simulink library "thermalCoupledCellResolution"  (R2025a)
settings: Solver=VariableStepAuto  StartTime=0.0  StopTime=10.0  RelTol=1e-3
undefined symbols (not defined in the file or in its folder): battery_builder_rtmsupport, gcbh
libraries: thermalCoupledCellResolution_lib x32
(part 2 of 3)

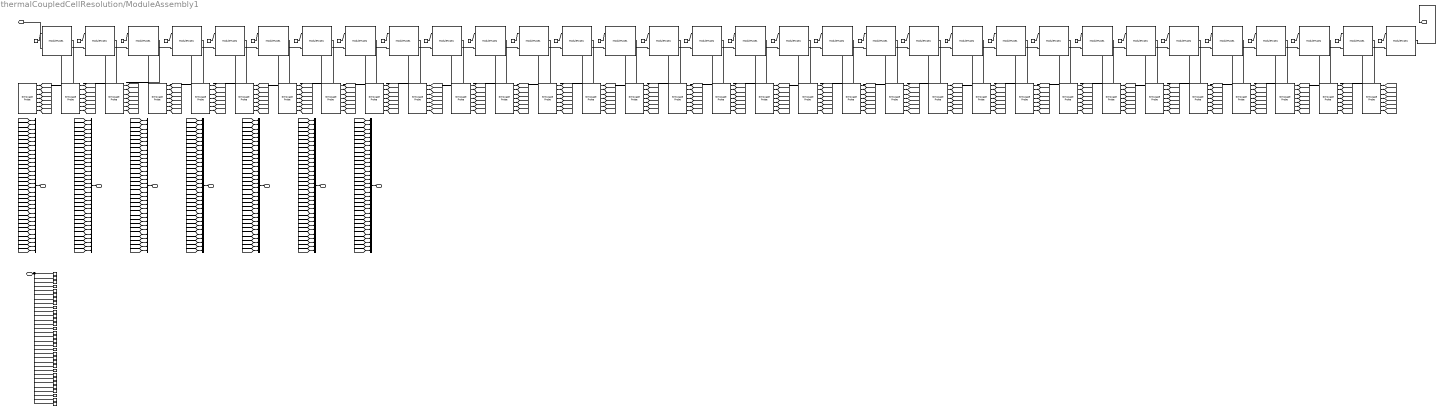
== system thermalCoupledCellResolution/ModuleAssembly1 ==
  note: Battery Modules
  note: Output Signals
  note: Thermal Boundary Conditions
  AmbH_From_1 : ConnectionLabel  Label=ambH_1
  AmbH_From_10 : ConnectionLabel  Label=ambH_10
  AmbH_From_11 : ConnectionLabel  Label=ambH_11
  AmbH_From_12 : ConnectionLabel  Label=ambH_12
  AmbH_From_13 : ConnectionLabel  Label=ambH_13
  AmbH_From_14 : ConnectionLabel  Label=ambH_14
  AmbH_From_15 : ConnectionLabel  Label=ambH_15
  AmbH_From_16 : ConnectionLabel  Label=ambH_16
  AmbH_From_17 : ConnectionLabel  Label=ambH_17
  AmbH_From_18 : ConnectionLabel  Label=ambH_18
  AmbH_From_19 : ConnectionLabel  Label=ambH_19
  AmbH_From_2 : ConnectionLabel  Label=ambH_2
  AmbH_From_20 : ConnectionLabel  Label=ambH_20
  AmbH_From_21 : ConnectionLabel  Label=ambH_21
  AmbH_From_22 : ConnectionLabel  Label=ambH_22
  AmbH_From_23 : ConnectionLabel  Label=ambH_23
  AmbH_From_24 : ConnectionLabel  Label=ambH_24
  AmbH_From_25 : ConnectionLabel  Label=ambH_25
  AmbH_From_26 : ConnectionLabel  Label=ambH_26
  AmbH_From_27 : ConnectionLabel  Label=ambH_27
  AmbH_From_28 : ConnectionLabel  Label=ambH_28
  AmbH_From_29 : ConnectionLabel  Label=ambH_29
  AmbH_From_3 : ConnectionLabel  Label=ambH_3
  AmbH_From_30 : ConnectionLabel  Label=ambH_30
  AmbH_From_31 : ConnectionLabel  Label=ambH_31
  AmbH_From_32 : ConnectionLabel  Label=ambH_32
  AmbH_From_4 : ConnectionLabel  Label=ambH_4
  AmbH_From_5 : ConnectionLabel  Label=ambH_5
  AmbH_From_6 : ConnectionLabel  Label=ambH_6
  AmbH_From_7 : ConnectionLabel  Label=ambH_7
  AmbH_From_8 : ConnectionLabel  Label=ambH_8
  AmbH_From_9 : ConnectionLabel  Label=ambH_9
  AmbH_To_1 : ConnectionLabel  Label=ambH_1
  AmbH_To_10 : ConnectionLabel  Label=ambH_10
  AmbH_To_11 : ConnectionLabel  Label=ambH_11
  AmbH_To_12 : ConnectionLabel  Label=ambH_12
  AmbH_To_13 : ConnectionLabel  Label=ambH_13
  AmbH_To_14 : ConnectionLabel  Label=ambH_14
  AmbH_To_15 : ConnectionLabel  Label=ambH_15
  AmbH_To_16 : ConnectionLabel  Label=ambH_16
  AmbH_To_17 : ConnectionLabel  Label=ambH_17
  AmbH_To_18 : ConnectionLabel  Label=ambH_18
  AmbH_To_19 : ConnectionLabel  Label=ambH_19
  AmbH_To_2 : ConnectionLabel  Label=ambH_2
  AmbH_To_20 : ConnectionLabel  Label=ambH_20
  AmbH_To_21 : ConnectionLabel  Label=ambH_21
  AmbH_To_22 : ConnectionLabel  Label=ambH_22
  AmbH_To_23 : ConnectionLabel  Label=ambH_23
  AmbH_To_24 : ConnectionLabel  Label=ambH_24
  AmbH_To_25 : ConnectionLabel  Label=ambH_25
  AmbH_To_26 : ConnectionLabel  Label=ambH_26
  AmbH_To_27 : ConnectionLabel  Label=ambH_27
  AmbH_To_28 : ConnectionLabel  Label=ambH_28
  AmbH_To_29 : ConnectionLabel  Label=ambH_29
  AmbH_To_3 : ConnectionLabel  Label=ambH_3
  AmbH_To_30 : ConnectionLabel  Label=ambH_30
  AmbH_To_31 : ConnectionLabel  Label=ambH_31
  AmbH_To_32 : ConnectionLabel  Label=ambH_32
  AmbH_To_4 : ConnectionLabel  Label=ambH_4
  AmbH_To_5 : ConnectionLabel  Label=ambH_5
  AmbH_To_6 : ConnectionLabel  Label=ambH_6
  AmbH_To_7 : ConnectionLabel  Label=ambH_7
  AmbH_To_8 : ConnectionLabel  Label=ambH_8
  AmbH_To_9 : ConnectionLabel  Label=ambH_9
  Module01 : thermalCoupledCellResolution_lib/Modules/ModuleType1  BatteryCapacityCell=Module01.BatteryCapacityCell A*hr  BatteryCapacityCellPercentDeviation=Module01.BatteryCapacityCellPercentDeviation  ExtrapolationMethodCell=simscape.enum.extrapolation.nearest  SOCBreakpointsCell=Module01.SOCBreakpointsCell  SOCBreakpointsCellPercentDeviation=Module01.SOCBreakpointsCellPercentDeviation  TemperatureBreakpointsCell=Module01.TemperatureBreakpointsCell K  TemperatureBreakpointsCellPercentDeviation=Module01.TemperatureBreakpointsCellPercentDeviation  OpenCircuitVoltageThermalCell=Module01.OpenCircuitVoltageThermalCell V  OpenCircuitVoltageThermalCellPercentDeviation=Module01.OpenCircuitVoltageThermalCellPercentDeviation  VoltageRangeCell=Module01.VoltageRangeCell V  VoltageRangeCellPercentDeviation=Module01.VoltageRangeCellPercentDeviation  ResistanceSOCBreakpointsCell=Module01.ResistanceSOCBreakpointsCell  ResistanceSOCBreakpointsCellPercentDeviation=Module01.ResistanceSOCBreakpointsCellPercentDeviation  ResistanceTemperatureBreakpointsCell=Module01.ResistanceTemperatureBreakpointsCell K  ResistanceTemperatureBreakpointsCellPercentDeviation=Module01.ResistanceTemperatureBreakpointsCellPercentDeviation  R0ThermalCell=Module01.R0ThermalCell Ohm  R0ThermalCellPercentDeviation=Module01.R0ThermalCellPercentDeviation  R1ThermalCell=Module01.R1ThermalCell Ohm  R1ThermalCellPercentDeviation=Module01.R1ThermalCellPercentDeviation  Tau1ThermalCell=Module01.Tau1ThermalCell s  Tau1ThermalCellPercentDeviation=Module01.Tau1ThermalCellPercentDeviation  BatteryThermalMassCell=Module01.BatteryThermalMassCell J/K  BatteryThermalMassCellPercentDeviation=Module01.BatteryThermalMassCellPercentDeviation  AmbientResistance=Module01.AmbientResistance K/W  P=2  S=6  socCell_specify=on  socCell_priority=High  socCell=Module01.socCell  socCell_nominal_specify=off  socCell_nominal_value=1  socCell_nominal_unit=1  batteryVoltage_specify=on  batteryVoltage_priority=None  batteryVoltage=Module01.batteryVoltage V  batteryVoltage_nominal_specify=off  batteryVoltage_nominal_value=1  batteryVoltage_nominal_unit=V  batteryCurrent_specify=on  batteryCurrent_priority=None  batteryCurrent=Module01.batteryCurrent A  batteryCurrent_nominal_specify=off  batteryCurrent_nominal_value=1  batteryCurrent_nominal_unit=A  numCycles_specify=on  numCycles_priority=High  numCycles=Module01.numCycles  numCycles_nominal_specify=off  numCycles_nominal_value=1  numCycles_nominal_unit=1  batteryTemperature_specify=on  batteryTemperature_priority=High  batteryTemperature=Module01.batteryTemperature K  batteryTemperature_nominal_specify=off  batteryTemperature_nominal_value=1  batteryTemperature_nominal_unit=K  vParallelAssembly_specify=on  vParallelAssembly_priority=None  vParallelAssembly=Module01.vParallelAssembly V  vParallelAssembly_nominal_specify=off  vParallelAssembly_nominal_value=1  vParallelAssembly_nominal_unit=V  socParallelAssembly_specify=on  socParallelAssembly_priority=None  socParallelAssembly=Module01.socParallelAssembly  socParallelAssembly_nominal_specify=off  socParallelAssembly_nominal_value=1  socParallelAssembly_nominal_unit=1
      settings: InternalSimscapePortConfiguration="{\"Bottom\":[{\"id\":\"n\",\"label\":\"-\",\"type\":\"foundation.electrical.electrical\"}],\"Left\":[{\"id\":\"AmbH\",\"label\":\"AmbH\",\"type\":\"foundation.thermal.thermal\"}],\"Right\":[],\"Top\":[{\"id\":\"p\",\"label\":\"+\",\"type\":\"foundation.electrical.electrical\"}]}"
  Module01_outputs : SimscapeProbe  BoundBlock=2  Variables="{\"batteryCurrent\":{\"Probing\":\"ON\"},\"batteryTemperature\":{\"Probing\":\"ON\"},\"batteryVoltage\":{\"Probing\":\"ON\"},\"numCycles\":{\"Probing\":\"ON\"},\"socCell\":{\"Probing\":\"ON\"},\"socParallelAssembly\":{\"Probing\":\"ON\"},\"vParallelAssembly\":{\"Probing\":\"ON\"}}"
  Module02 : thermalCoupledCellResolution_lib/Modules/ModuleType1  BatteryCapacityCell=Module02.BatteryCapacityCell A*hr  BatteryCapacityCellPercentDeviation=Module02.BatteryCapacityCellPercentDeviation  ExtrapolationMethodCell=simscape.enum.extrapolation.nearest  SOCBreakpointsCell=Module02.SOCBreakpointsCell  SOCBreakpointsCellPercentDeviation=Module02.SOCBreakpointsCellPercentDeviation  TemperatureBreakpointsCell=Module02.TemperatureBreakpointsCell K  TemperatureBreakpointsCellPercentDeviation=Module02.TemperatureBreakpointsCellPercentDeviation  OpenCircuitVoltageThermalCell=Module02.OpenCircuitVoltageThermalCell V  OpenCircuitVoltageThermalCellPercentDeviation=Module02.OpenCircuitVoltageThermalCellPercentDeviation  VoltageRangeCell=Module02.VoltageRangeCell V  VoltageRangeCellPercentDeviation=Module02.VoltageRangeCellPercentDeviation  ResistanceSOCBreakpointsCell=Module02.ResistanceSOCBreakpointsCell  ResistanceSOCBreakpointsCellPercentDeviation=Module02.ResistanceSOCBreakpointsCellPercentDeviation  ResistanceTemperatureBreakpointsCell=Module02.ResistanceTemperatureBreakpointsCell K  ResistanceTemperatureBreakpointsCellPercentDeviation=Module02.ResistanceTemperatureBreakpointsCellPercentDeviation  R0ThermalCell=Module02.R0ThermalCell Ohm  R0ThermalCellPercentDeviation=Module02.R0ThermalCellPercentDeviation  R1ThermalCell=Module02.R1ThermalCell Ohm  R1ThermalCellPercentDeviation=Module02.R1ThermalCellPercentDeviation  Tau1ThermalCell=Module02.Tau1ThermalCell s  Tau1ThermalCellPercentDeviation=Module02.Tau1ThermalCellPercentDeviation  BatteryThermalMassCell=Module02.BatteryThermalMassCell J/K  BatteryThermalMassCellPercentDeviation=Module02.BatteryThermalMassCellPercentDeviation  AmbientResistance=Module02.AmbientResistance K/W  P=2  S=6  socCell_specify=on  socCell_priority=High  socCell=Module02.socCell  socCell_nominal_specify=off  socCell_nominal_value=1  socCell_nominal_unit=1  batteryVoltage_specify=on  batteryVoltage_priority=None  batteryVoltage=Module02.batteryVoltage V  batteryVoltage_nominal_specify=off  batteryVoltage_nominal_value=1  batteryVoltage_nominal_unit=V  batteryCurrent_specify=on  batteryCurrent_priority=None  batteryCurrent=Module02.batteryCurrent A  batteryCurrent_nominal_specify=off  batteryCurrent_nominal_value=1  batteryCurrent_nominal_unit=A  numCycles_specify=on  numCycles_priority=High  numCycles=Module02.numCycles  numCycles_nominal_specify=off  numCycles_nominal_value=1  numCycles_nominal_unit=1  batteryTemperature_specify=on  batteryTemperature_priority=High  batteryTemperature=Module02.batteryTemperature K  batteryTemperature_nominal_specify=off  batteryTemperature_nominal_value=1  batteryTemperature_nominal_unit=K  vParallelAssembly_specify=on  vParallelAssembly_priority=None  vParallelAssembly=Module02.vParallelAssembly V  vParallelAssembly_nominal_specify=off  vParallelAssembly_nominal_value=1  vParallelAssembly_nominal_unit=V  socParallelAssembly_specify=on  socParallelAssembly_priority=None  socParallelAssembly=Module02.socParallelAssembly  socParallelAssembly_nominal_specify=off  socParallelAssembly_nominal_value=1  socParallelAssembly_nominal_unit=1
      settings: InternalSimscapePortConfiguration="{\"Bottom\":[{\"id\":\"n\",\"label\":\"-\",\"type\":\"foundation.electrical.electrical\"}],\"Left\":[{\"id\":\"AmbH\",\"label\":\"AmbH\",\"type\":\"foundation.thermal.thermal\"}],\"Right\":[],\"Top\":[{\"id\":\"p\",\"label\":\"+\",\"type\":\"foundation.electrical.electrical\"}]}"
  Module02_outputs : SimscapeProbe  BoundBlock=3  Variables="{\"batteryCurrent\":{\"Probing\":\"ON\"},\"batteryTemperature\":{\"Probing\":\"ON\"},\"batteryVoltage\":{\"Probing\":\"ON\"},\"numCycles\":{\"Probing\":\"ON\"},\"socCell\":{\"Probing\":\"ON\"},\"socParallelAssembly\":{\"Probing\":\"ON\"},\"vParallelAssembly\":{\"Probing\":\"ON\"}}"
  Module03 : thermalCoupledCellResolution_lib/Modules/ModuleType1  BatteryCapacityCell=Module03.BatteryCapacityCell A*hr  BatteryCapacityCellPercentDeviation=Module03.BatteryCapacityCellPercentDeviation  ExtrapolationMethodCell=simscape.enum.extrapolation.nearest  SOCBreakpointsCell=Module03.SOCBreakpointsCell  SOCBreakpointsCellPercentDeviation=Module03.SOCBreakpointsCellPercentDeviation  TemperatureBreakpointsCell=Module03.TemperatureBreakpointsCell K  TemperatureBreakpointsCellPercentDeviation=Module03.TemperatureBreakpointsCellPercentDeviation  OpenCircuitVoltageThermalCell=Module03.OpenCircuitVoltageThermalCell V  OpenCircuitVoltageThermalCellPercentDeviation=Module03.OpenCircuitVoltageThermalCellPercentDeviation  VoltageRangeCell=Module03.VoltageRangeCell V  VoltageRangeCellPercentDeviation=Module03.VoltageRangeCellPercentDeviation  ResistanceSOCBreakpointsCell=Module03.ResistanceSOCBreakpointsCell  ResistanceSOCBreakpointsCellPercentDeviation=Module03.ResistanceSOCBreakpointsCellPercentDeviation  ResistanceTemperatureBreakpointsCell=Module03.ResistanceTemperatureBreakpointsCell K  ResistanceTemperatureBreakpointsCellPercentDeviation=Module03.ResistanceTemperatureBreakpointsCellPercentDeviation  R0ThermalCell=Module03.R0ThermalCell Ohm  R0ThermalCellPercentDeviation=Module03.R0ThermalCellPercentDeviation  R1ThermalCell=Module03.R1ThermalCell Ohm  R1ThermalCellPercentDeviation=Module03.R1ThermalCellPercentDeviation  Tau1ThermalCell=Module03.Tau1ThermalCell s  Tau1ThermalCellPercentDeviation=Module03.Tau1ThermalCellPercentDeviation  BatteryThermalMassCell=Module03.BatteryThermalMassCell J/K  BatteryThermalMassCellPercentDeviation=Module03.BatteryThermalMassCellPercentDeviation  AmbientResistance=Module03.AmbientResistance K/W  P=2  S=6  socCell_specify=on  socCell_priority=High  socCell=Module03.socCell  socCell_nominal_specify=off  socCell_nominal_value=1  socCell_nominal_unit=1  batteryVoltage_specify=on  batteryVoltage_priority=None  batteryVoltage=Module03.batteryVoltage V  batteryVoltage_nominal_specify=off  batteryVoltage_nominal_value=1  batteryVoltage_nominal_unit=V  batteryCurrent_specify=on  batteryCurrent_priority=None  batteryCurrent=Module03.batteryCurrent A  batteryCurrent_nominal_specify=off  batteryCurrent_nominal_value=1  batteryCurrent_nominal_unit=A  numCycles_specify=on  numCycles_priority=High  numCycles=Module03.numCycles  numCycles_nominal_specify=off  numCycles_nominal_value=1  numCycles_nominal_unit=1  batteryTemperature_specify=on  batteryTemperature_priority=High  batteryTemperature=Module03.batteryTemperature K  batteryTemperature_nominal_specify=off  batteryTemperature_nominal_value=1  batteryTemperature_nominal_unit=K  vParallelAssembly_specify=on  vParallelAssembly_priority=None  vParallelAssembly=Module03.vParallelAssembly V  vParallelAssembly_nominal_specify=off  vParallelAssembly_nominal_value=1  vParallelAssembly_nominal_unit=V  socParallelAssembly_specify=on  socParallelAssembly_priority=None  socParallelAssembly=Module03.socParallelAssembly  socParallelAssembly_nominal_specify=off  socParallelAssembly_nominal_value=1  socParallelAssembly_nominal_unit=1
      settings: InternalSimscapePortConfiguration="{\"Bottom\":[{\"id\":\"n\",\"label\":\"-\",\"type\":\"foundation.electrical.electrical\"}],\"Left\":[{\"id\":\"AmbH\",\"label\":\"AmbH\",\"type\":\"foundation.thermal.thermal\"}],\"Right\":[],\"Top\":[{\"id\":\"p\",\"label\":\"+\",\"type\":\"foundation.electrical.electrical\"}]}"
  Module03_outputs : SimscapeProbe  BoundBlock=4  Variables="{\"batteryCurrent\":{\"Probing\":\"ON\"},\"batteryTemperature\":{\"Probing\":\"ON\"},\"batteryVoltage\":{\"Probing\":\"ON\"},\"numCycles\":{\"Probing\":\"ON\"},\"socCell\":{\"Probing\":\"ON\"},\"socParallelAssembly\":{\"Probing\":\"ON\"},\"vParallelAssembly\":{\"Probing\":\"ON\"}}"
  Module04 : thermalCoupledCellResolution_lib/Modules/ModuleType1  BatteryCapacityCell=Module04.BatteryCapacityCell A*hr  BatteryCapacityCellPercentDeviation=Module04.BatteryCapacityCellPercentDeviation  ExtrapolationMethodCell=simscape.enum.extrapolation.nearest  SOCBreakpointsCell=Module04.SOCBreakpointsCell  SOCBreakpointsCellPercentDeviation=Module04.SOCBreakpointsCellPercentDeviation  TemperatureBreakpointsCell=Module04.TemperatureBreakpointsCell K  TemperatureBreakpointsCellPercentDeviation=Module04.TemperatureBreakpointsCellPercentDeviation  OpenCircuitVoltageThermalCell=Module04.OpenCircuitVoltageThermalCell V  OpenCircuitVoltageThermalCellPercentDeviation=Module04.OpenCircuitVoltageThermalCellPercentDeviation  VoltageRangeCell=Module04.VoltageRangeCell V  VoltageRangeCellPercentDeviation=Module04.VoltageRangeCellPercentDeviation  ResistanceSOCBreakpointsCell=Module04.ResistanceSOCBreakpointsCell  ResistanceSOCBreakpointsCellPercentDeviation=Module04.ResistanceSOCBreakpointsCellPercentDeviation  ResistanceTemperatureBreakpointsCell=Module04.ResistanceTemperatureBreakpointsCell K  ResistanceTemperatureBreakpointsCellPercentDeviation=Module04.ResistanceTemperatureBreakpointsCellPercentDeviation  R0ThermalCell=Module04.R0ThermalCell Ohm  R0ThermalCellPercentDeviation=Module04.R0ThermalCellPercentDeviation  R1ThermalCell=Module04.R1ThermalCell Ohm  R1ThermalCellPercentDeviation=Module04.R1ThermalCellPercentDeviation  Tau1ThermalCell=Module04.Tau1ThermalCell s  Tau1ThermalCellPercentDeviation=Module04.Tau1ThermalCellPercentDeviation  BatteryThermalMassCell=Module04.BatteryThermalMassCell J/K  BatteryThermalMassCellPercentDeviation=Module04.BatteryThermalMassCellPercentDeviation  AmbientResistance=Module04.AmbientResistance K/W  P=2  S=6  socCell_specify=on  socCell_priority=High  socCell=Module04.socCell  socCell_nominal_specify=off  socCell_nominal_value=1  socCell_nominal_unit=1  batteryVoltage_specify=on  batteryVoltage_priority=None  batteryVoltage=Module04.batteryVoltage V  batteryVoltage_nominal_specify=off  batteryVoltage_nominal_value=1  batteryVoltage_nominal_unit=V  batteryCurrent_specify=on  batteryCurrent_priority=None  batteryCurrent=Module04.batteryCurrent A  batteryCurrent_nominal_specify=off  batteryCurrent_nominal_value=1  batteryCurrent_nominal_unit=A  numCycles_specify=on  numCycles_priority=High  numCycles=Module04.numCycles  numCycles_nominal_specify=off  numCycles_nominal_value=1  numCycles_nominal_unit=1  batteryTemperature_specify=on  batteryTemperature_priority=High  batteryTemperature=Module04.batteryTemperature K  batteryTemperature_nominal_specify=off  batteryTemperature_nominal_value=1  batteryTemperature_nominal_unit=K  vParallelAssembly_specify=on  vParallelAssembly_priority=None  vParallelAssembly=Module04.vParallelAssembly V  vParallelAssembly_nominal_specify=off  vParallelAssembly_nominal_value=1  vParallelAssembly_nominal_unit=V  socParallelAssembly_specify=on  socParallelAssembly_priority=None  socParallelAssembly=Module04.socParallelAssembly  socParallelAssembly_nominal_specify=off  socParallelAssembly_nominal_value=1  socParallelAssembly_nominal_unit=1
      settings: InternalSimscapePortConfiguration="{\"Bottom\":[{\"id\":\"n\",\"label\":\"-\",\"type\":\"foundation.electrical.electrical\"}],\"Left\":[{\"id\":\"AmbH\",\"label\":\"AmbH\",\"type\":\"foundation.thermal.thermal\"}],\"Right\":[],\"Top\":[{\"id\":\"p\",\"label\":\"+\",\"type\":\"foundation.electrical.electrical\"}]}"
  Module04_outputs : SimscapeProbe  BoundBlock=5  Variables="{\"batteryCurrent\":{\"Probing\":\"ON\"},\"batteryTemperature\":{\"Probing\":\"ON\"},\"batteryVoltage\":{\"Probing\":\"ON\"},\"numCycles\":{\"Probing\":\"ON\"},\"socCell\":{\"Probing\":\"ON\"},\"socParallelAssembly\":{\"Probing\":\"ON\"},\"vParallelAssembly\":{\"Probing\":\"ON\"}}"
  Module05 : thermalCoupledCellResolution_lib/Modules/ModuleType1  BatteryCapacityCell=Module05.BatteryCapacityCell A*hr  BatteryCapacityCellPercentDeviation=Module05.BatteryCapacityCellPercentDeviation  ExtrapolationMethodCell=simscape.enum.extrapolation.nearest  SOCBreakpointsCell=Module05.SOCBreakpointsCell  SOCBreakpointsCellPercentDeviation=Module05.SOCBreakpointsCellPercentDeviation  TemperatureBreakpointsCell=Module05.TemperatureBreakpointsCell K  TemperatureBreakpointsCellPercentDeviation=Module05.TemperatureBreakpointsCellPercentDeviation  OpenCircuitVoltageThermalCell=Module05.OpenCircuitVoltageThermalCell V  OpenCircuitVoltageThermalCellPercentDeviation=Module05.OpenCircuitVoltageThermalCellPercentDeviation  VoltageRangeCell=Module05.VoltageRangeCell V  VoltageRangeCellPercentDeviation=Module05.VoltageRangeCellPercentDeviation  ResistanceSOCBreakpointsCell=Module05.ResistanceSOCBreakpointsCell  ResistanceSOCBreakpointsCellPercentDeviation=Module05.ResistanceSOCBreakpointsCellPercentDeviation  ResistanceTemperatureBreakpointsCell=Module05.ResistanceTemperatureBreakpointsCell K  ResistanceTemperatureBreakpointsCellPercentDeviation=Module05.ResistanceTemperatureBreakpointsCellPercentDeviation  R0ThermalCell=Module05.R0ThermalCell Ohm  R0ThermalCellPercentDeviation=Module05.R0ThermalCellPercentDeviation  R1ThermalCell=Module05.R1ThermalCell Ohm  R1ThermalCellPercentDeviation=Module05.R1ThermalCellPercentDeviation  Tau1ThermalCell=Module05.Tau1ThermalCell s  Tau1ThermalCellPercentDeviation=Module05.Tau1ThermalCellPercentDeviation  BatteryThermalMassCell=Module05.BatteryThermalMassCell J/K  BatteryThermalMassCellPercentDeviation=Module05.BatteryThermalMassCellPercentDeviation  AmbientResistance=Module05.AmbientResistance K/W  P=2  S=6  socCell_specify=on  socCell_priority=High  socCell=Module05.socCell  socCell_nominal_specify=off  socCell_nominal_value=1  socCell_nominal_unit=1  batteryVoltage_specify=on  batteryVoltage_priority=None  batteryVoltage=Module05.batteryVoltage V  batteryVoltage_nominal_specify=off  batteryVoltage_nominal_value=1  batteryVoltage_nominal_unit=V  batteryCurrent_specify=on  batteryCurrent_priority=None  batteryCurrent=Module05.batteryCurrent A  batteryCurrent_nominal_specify=off  batteryCurrent_nominal_value=1  batteryCurrent_nominal_unit=A  numCycles_specify=on  numCycles_priority=High  numCycles=Module05.numCycles  numCycles_nominal_specify=off  numCycles_nominal_value=1  numCycles_nominal_unit=1  batteryTemperature_specify=on  batteryTemperature_priority=High  batteryTemperature=Module05.batteryTemperature K  batteryTemperature_nominal_specify=off  batteryTemperature_nominal_value=1  batteryTemperature_nominal_unit=K  vParallelAssembly_specify=on  vParallelAssembly_priority=None  vParallelAssembly=Module05.vParallelAssembly V  vParallelAssembly_nominal_specify=off  vParallelAssembly_nominal_value=1  vParallelAssembly_nominal_unit=V  socParallelAssembly_specify=on  socParallelAssembly_priority=None  socParallelAssembly=Module05.socParallelAssembly  socParallelAssembly_nominal_specify=off  socParallelAssembly_nominal_value=1  socParallelAssembly_nominal_unit=1
      settings: InternalSimscapePortConfiguration="{\"Bottom\":[{\"id\":\"n\",\"label\":\"-\",\"type\":\"foundation.electrical.electrical\"}],\"Left\":[{\"id\":\"AmbH\",\"label\":\"AmbH\",\"type\":\"foundation.thermal.thermal\"}],\"Right\":[],\"Top\":[{\"id\":\"p\",\"label\":\"+\",\"type\":\"foundation.electrical.electrical\"}]}"
  Module05_outputs : SimscapeProbe  BoundBlock=6  Variables="{\"batteryCurrent\":{\"Probing\":\"ON\"},\"batteryTemperature\":{\"Probing\":\"ON\"},\"batteryVoltage\":{\"Probing\":\"ON\"},\"numCycles\":{\"Probing\":\"ON\"},\"socCell\":{\"Probing\":\"ON\"},\"socParallelAssembly\":{\"Probing\":\"ON\"},\"vParallelAssembly\":{\"Probing\":\"ON\"}}"
  Module06 : thermalCoupledCellResolution_lib/Modules/ModuleType1  BatteryCapacityCell=Module06.BatteryCapacityCell A*hr  BatteryCapacityCellPercentDeviation=Module06.BatteryCapacityCellPercentDeviation  ExtrapolationMethodCell=simscape.enum.extrapolation.nearest  SOCBreakpointsCell=Module06.SOCBreakpointsCell  SOCBreakpointsCellPercentDeviation=Module06.SOCBreakpointsCellPercentDeviation  TemperatureBreakpointsCell=Module06.TemperatureBreakpointsCell K  TemperatureBreakpointsCellPercentDeviation=Module06.TemperatureBreakpointsCellPercentDeviation  OpenCircuitVoltageThermalCell=Module06.OpenCircuitVoltageThermalCell V  OpenCircuitVoltageThermalCellPercentDeviation=Module06.OpenCircuitVoltageThermalCellPercentDeviation  VoltageRangeCell=Module06.VoltageRangeCell V  VoltageRangeCellPercentDeviation=Module06.VoltageRangeCellPercentDeviation  ResistanceSOCBreakpointsCell=Module06.ResistanceSOCBreakpointsCell  ResistanceSOCBreakpointsCellPercentDeviation=Module06.ResistanceSOCBreakpointsCellPercentDeviation  ResistanceTemperatureBreakpointsCell=Module06.ResistanceTemperatureBreakpointsCell K  ResistanceTemperatureBreakpointsCellPercentDeviation=Module06.ResistanceTemperatureBreakpointsCellPercentDeviation  R0ThermalCell=Module06.R0ThermalCell Ohm  R0ThermalCellPercentDeviation=Module06.R0ThermalCellPercentDeviation  R1ThermalCell=Module06.R1ThermalCell Ohm  R1ThermalCellPercentDeviation=Module06.R1ThermalCellPercentDeviation  Tau1ThermalCell=Module06.Tau1ThermalCell s  Tau1ThermalCellPercentDeviation=Module06.Tau1ThermalCellPercentDeviation  BatteryThermalMassCell=Module06.BatteryThermalMassCell J/K  BatteryThermalMassCellPercentDeviation=Module06.BatteryThermalMassCellPercentDeviation  AmbientResistance=Module06.AmbientResistance K/W  P=2  S=6  socCell_specify=on  socCell_priority=High  socCell=Module06.socCell  socCell_nominal_specify=off  socCell_nominal_value=1  socCell_nominal_unit=1  batteryVoltage_specify=on  batteryVoltage_priority=None  batteryVoltage=Module06.batteryVoltage V  batteryVoltage_nominal_specify=off  batteryVoltage_nominal_value=1  batteryVoltage_nominal_unit=V  batteryCurrent_specify=on  batteryCurrent_priority=None  batteryCurrent=Module06.batteryCurrent A  batteryCurrent_nominal_specify=off  batteryCurrent_nominal_value=1  batteryCurrent_nominal_unit=A  numCycles_specify=on  numCycles_priority=High  numCycles=Module06.numCycles  numCycles_nominal_specify=off  numCycles_nominal_value=1  numCycles_nominal_unit=1  batteryTemperature_specify=on  batteryTemperature_priority=High  batteryTemperature=Module06.batteryTemperature K  batteryTemperature_nominal_specify=off  batteryTemperature_nominal_value=1  batteryTemperature_nominal_unit=K  vParallelAssembly_specify=on  vParallelAssembly_priority=None  vParallelAssembly=Module06.vParallelAssembly V  vParallelAssembly_nominal_specify=off  vParallelAssembly_nominal_value=1  vParallelAssembly_nominal_unit=V  socParallelAssembly_specify=on  socParallelAssembly_priority=None  socParallelAssembly=Module06.socParallelAssembly  socParallelAssembly_nominal_specify=off  socParallelAssembly_nominal_value=1  socParallelAssembly_nominal_unit=1
      settings: InternalSimscapePortConfiguration="{\"Bottom\":[{\"id\":\"n\",\"label\":\"-\",\"type\":\"foundation.electrical.electrical\"}],\"Left\":[{\"id\":\"AmbH\",\"label\":\"AmbH\",\"type\":\"foundation.thermal.thermal\"}],\"Right\":[],\"Top\":[{\"id\":\"p\",\"label\":\"+\",\"type\":\"foundation.electrical.electrical\"}]}"
  Module06_outputs : SimscapeProbe  BoundBlock=7  Variables="{\"batteryCurrent\":{\"Probing\":\"ON\"},\"batteryTemperature\":{\"Probing\":\"ON\"},\"batteryVoltage\":{\"Probing\":\"ON\"},\"numCycles\":{\"Probing\":\"ON\"},\"socCell\":{\"Probing\":\"ON\"},\"socParallelAssembly\":{\"Probing\":\"ON\"},\"vParallelAssembly\":{\"Probing\":\"ON\"}}"
  Module07 : thermalCoupledCellResolution_lib/Modules/ModuleType1  BatteryCapacityCell=Module07.BatteryCapacityCell A*hr  BatteryCapacityCellPercentDeviation=Module07.BatteryCapacityCellPercentDeviation  ExtrapolationMethodCell=simscape.enum.extrapolation.nearest  SOCBreakpointsCell=Module07.SOCBreakpointsCell  SOCBreakpointsCellPercentDeviation=Module07.SOCBreakpointsCellPercentDeviation  TemperatureBreakpointsCell=Module07.TemperatureBreakpointsCell K  TemperatureBreakpointsCellPercentDeviation=Module07.TemperatureBreakpointsCellPercentDeviation  OpenCircuitVoltageThermalCell=Module07.OpenCircuitVoltageThermalCell V  OpenCircuitVoltageThermalCellPercentDeviation=Module07.OpenCircuitVoltageThermalCellPercentDeviation  VoltageRangeCell=Module07.VoltageRangeCell V  VoltageRangeCellPercentDeviation=Module07.VoltageRangeCellPercentDeviation  ResistanceSOCBreakpointsCell=Module07.ResistanceSOCBreakpointsCell  ResistanceSOCBreakpointsCellPercentDeviation=Module07.ResistanceSOCBreakpointsCellPercentDeviation  ResistanceTemperatureBreakpointsCell=Module07.ResistanceTemperatureBreakpointsCell K  ResistanceTemperatureBreakpointsCellPercentDeviation=Module07.ResistanceTemperatureBreakpointsCellPercentDeviation  R0ThermalCell=Module07.R0ThermalCell Ohm  R0ThermalCellPercentDeviation=Module07.R0ThermalCellPercentDeviation  R1ThermalCell=Module07.R1ThermalCell Ohm  R1ThermalCellPercentDeviation=Module07.R1ThermalCellPercentDeviation  Tau1ThermalCell=Module07.Tau1ThermalCell s  Tau1ThermalCellPercentDeviation=Module07.Tau1ThermalCellPercentDeviation  BatteryThermalMassCell=Module07.BatteryThermalMassCell J/K  BatteryThermalMassCellPercentDeviation=Module07.BatteryThermalMassCellPercentDeviation  AmbientResistance=Module07.AmbientResistance K/W  P=2  S=6  socCell_specify=on  socCell_priority=High  socCell=Module07.socCell  socCell_nominal_specify=off  socCell_nominal_value=1  socCell_nominal_unit=1  batteryVoltage_specify=on  batteryVoltage_priority=None  batteryVoltage=Module07.batteryVoltage V  batteryVoltage_nominal_specify=off  batteryVoltage_nominal_value=1  batteryVoltage_nominal_unit=V  batteryCurrent_specify=on  batteryCurrent_priority=None  batteryCurrent=Module07.batteryCurrent A  batteryCurrent_nominal_specify=off  batteryCurrent_nominal_value=1  batteryCurrent_nominal_unit=A  numCycles_specify=on  numCycles_priority=High  numCycles=Module07.numCycles  numCycles_nominal_specify=off  numCycles_nominal_value=1  numCycles_nominal_unit=1  batteryTemperature_specify=on  batteryTemperature_priority=High  batteryTemperature=Module07.batteryTemperature K  batteryTemperature_nominal_specify=off  batteryTemperature_nominal_value=1  batteryTemperature_nominal_unit=K  vParallelAssembly_specify=on  vParallelAssembly_priority=None  vParallelAssembly=Module07.vParallelAssembly V  vParallelAssembly_nominal_specify=off  vParallelAssembly_nominal_value=1  vParallelAssembly_nominal_unit=V  socParallelAssembly_specify=on  socParallelAssembly_priority=None  socParallelAssembly=Module07.socParallelAssembly  socParallelAssembly_nominal_specify=off  socParallelAssembly_nominal_value=1  socParallelAssembly_nominal_unit=1
      settings: InternalSimscapePortConfiguration="{\"Bottom\":[{\"id\":\"n\",\"label\":\"-\",\"type\":\"foundation.electrical.electrical\"}],\"Left\":[{\"id\":\"AmbH\",\"label\":\"AmbH\",\"type\":\"foundation.thermal.thermal\"}],\"Right\":[],\"Top\":[{\"id\":\"p\",\"label\":\"+\",\"type\":\"foundation.electrical.electrical\"}]}"
  Module07_outputs : SimscapeProbe  BoundBlock=8  Variables="{\"batteryCurrent\":{\"Probing\":\"ON\"},\"batteryTemperature\":{\"Probing\":\"ON\"},\"batteryVoltage\":{\"Probing\":\"ON\"},\"numCycles\":{\"Probing\":\"ON\"},\"socCell\":{\"Probing\":\"ON\"},\"socParallelAssembly\":{\"Probing\":\"ON\"},\"vParallelAssembly\":{\"Probing\":\"ON\"}}"
  Module08 : thermalCoupledCellResolution_lib/Modules/ModuleType1  BatteryCapacityCell=Module08.BatteryCapacityCell A*hr  BatteryCapacityCellPercentDeviation=Module08.BatteryCapacityCellPercentDeviation  ExtrapolationMethodCell=simscape.enum.extrapolation.nearest  SOCBreakpointsCell=Module08.SOCBreakpointsCell  SOCBreakpointsCellPercentDeviation=Module08.SOCBreakpointsCellPercentDeviation  TemperatureBreakpointsCell=Module08.TemperatureBreakpointsCell K  TemperatureBreakpointsCellPercentDeviation=Module08.TemperatureBreakpointsCellPercentDeviation  OpenCircuitVoltageThermalCell=Module08.OpenCircuitVoltageThermalCell V  OpenCircuitVoltageThermalCellPercentDeviation=Module08.OpenCircuitVoltageThermalCellPercentDeviation  VoltageRangeCell=Module08.VoltageRangeCell V  VoltageRangeCellPercentDeviation=Module08.VoltageRangeCellPercentDeviation  ResistanceSOCBreakpointsCell=Module08.ResistanceSOCBreakpointsCell  ResistanceSOCBreakpointsCellPercentDeviation=Module08.ResistanceSOCBreakpointsCellPercentDeviation  ResistanceTemperatureBreakpointsCell=Module08.ResistanceTemperatureBreakpointsCell K  ResistanceTemperatureBreakpointsCellPercentDeviation=Module08.ResistanceTemperatureBreakpointsCellPercentDeviation  R0ThermalCell=Module08.R0ThermalCell Ohm  R0ThermalCellPercentDeviation=Module08.R0ThermalCellPercentDeviation  R1ThermalCell=Module08.R1ThermalCell Ohm  R1ThermalCellPercentDeviation=Module08.R1ThermalCellPercentDeviation  Tau1ThermalCell=Module08.Tau1ThermalCell s  Tau1ThermalCellPercentDeviation=Module08.Tau1ThermalCellPercentDeviation  BatteryThermalMassCell=Module08.BatteryThermalMassCell J/K  BatteryThermalMassCellPercentDeviation=Module08.BatteryThermalMassCellPercentDeviation  AmbientResistance=Module08.AmbientResistance K/W  P=2  S=6  socCell_specify=on  socCell_priority=High  socCell=Module08.socCell  socCell_nominal_specify=off  socCell_nominal_value=1  socCell_nominal_unit=1  batteryVoltage_specify=on  batteryVoltage_priority=None  batteryVoltage=Module08.batteryVoltage V  batteryVoltage_nominal_specify=off  batteryVoltage_nominal_value=1  batteryVoltage_nominal_unit=V  batteryCurrent_specify=on  batteryCurrent_priority=None  batteryCurrent=Module08.batteryCurrent A  batteryCurrent_nominal_specify=off  batteryCurrent_nominal_value=1  batteryCurrent_nominal_unit=A  numCycles_specify=on  numCycles_priority=High  numCycles=Module08.numCycles  numCycles_nominal_specify=off  numCycles_nominal_value=1  numCycles_nominal_unit=1  batteryTemperature_specify=on  batteryTemperature_priority=High  batteryTemperature=Module08.batteryTemperature K  batteryTemperature_nominal_specify=off  batteryTemperature_nominal_value=1  batteryTemperature_nominal_unit=K  vParallelAssembly_specify=on  vParallelAssembly_priority=None  vParallelAssembly=Module08.vParallelAssembly V  vParallelAssembly_nominal_specify=off  vParallelAssembly_nominal_value=1  vParallelAssembly_nominal_unit=V  socParallelAssembly_specify=on  socParallelAssembly_priority=None  socParallelAssembly=Module08.socParallelAssembly  socParallelAssembly_nominal_specify=off  socParallelAssembly_nominal_value=1  socParallelAssembly_nominal_unit=1
      settings: InternalSimscapePortConfiguration="{\"Bottom\":[{\"id\":\"n\",\"label\":\"-\",\"type\":\"foundation.electrical.electrical\"}],\"Left\":[{\"id\":\"AmbH\",\"label\":\"AmbH\",\"type\":\"foundation.thermal.thermal\"}],\"Right\":[],\"Top\":[{\"id\":\"p\",\"label\":\"+\",\"type\":\"foundation.electrical.electrical\"}]}"
  Module08_outputs : SimscapeProbe  BoundBlock=9  Variables="{\"batteryCurrent\":{\"Probing\":\"ON\"},\"batteryTemperature\":{\"Probing\":\"ON\"},\"batteryVoltage\":{\"Probing\":\"ON\"},\"numCycles\":{\"Probing\":\"ON\"},\"socCell\":{\"Probing\":\"ON\"},\"socParallelAssembly\":{\"Probing\":\"ON\"},\"vParallelAssembly\":{\"Probing\":\"ON\"}}"
  Module09 : thermalCoupledCellResolution_lib/Modules/ModuleType1  BatteryCapacityCell=Module09.BatteryCapacityCell A*hr  BatteryCapacityCellPercentDeviation=Module09.BatteryCapacityCellPercentDeviation  ExtrapolationMethodCell=simscape.enum.extrapolation.nearest  SOCBreakpointsCell=Module09.SOCBreakpointsCell  SOCBreakpointsCellPercentDeviation=Module09.SOCBreakpointsCellPercentDeviation  TemperatureBreakpointsCell=Module09.TemperatureBreakpointsCell K  TemperatureBreakpointsCellPercentDeviation=Module09.TemperatureBreakpointsCellPercentDeviation  OpenCircuitVoltageThermalCell=Module09.OpenCircuitVoltageThermalCell V  OpenCircuitVoltageThermalCellPercentDeviation=Module09.OpenCircuitVoltageThermalCellPercentDeviation  VoltageRangeCell=Module09.VoltageRangeCell V  VoltageRangeCellPercentDeviation=Module09.VoltageRangeCellPercentDeviation  ResistanceSOCBreakpointsCell=Module09.ResistanceSOCBreakpointsCell  ResistanceSOCBreakpointsCellPercentDeviation=Module09.ResistanceSOCBreakpointsCellPercentDeviation  ResistanceTemperatureBreakpointsCell=Module09.ResistanceTemperatureBreakpointsCell K  ResistanceTemperatureBreakpointsCellPercentDeviation=Module09.ResistanceTemperatureBreakpointsCellPercentDeviation  R0ThermalCell=Module09.R0ThermalCell Ohm  R0ThermalCellPercentDeviation=Module09.R0ThermalCellPercentDeviation  R1ThermalCell=Module09.R1ThermalCell Ohm  R1ThermalCellPercentDeviation=Module09.R1ThermalCellPercentDeviation  Tau1ThermalCell=Module09.Tau1ThermalCell s  Tau1ThermalCellPercentDeviation=Module09.Tau1ThermalCellPercentDeviation  BatteryThermalMassCell=Module09.BatteryThermalMassCell J/K  BatteryThermalMassCellPercentDeviation=Module09.BatteryThermalMassCellPercentDeviation  AmbientResistance=Module09.AmbientResistance K/W  P=2  S=6  socCell_specify=on  socCell_priority=High  socCell=Module09.socCell  socCell_nominal_specify=off  socCell_nominal_value=1  socCell_nominal_unit=1  batteryVoltage_specify=on  batteryVoltage_priority=None  batteryVoltage=Module09.batteryVoltage V  batteryVoltage_nominal_specify=off  batteryVoltage_nominal_value=1  batteryVoltage_nominal_unit=V  batteryCurrent_specify=on  batteryCurrent_priority=None  batteryCurrent=Module09.batteryCurrent A  batteryCurrent_nominal_specify=off  batteryCurrent_nominal_value=1  batteryCurrent_nominal_unit=A  numCycles_specify=on  numCycles_priority=High  numCycles=Module09.numCycles  numCycles_nominal_specify=off  numCycles_nominal_value=1  numCycles_nominal_unit=1  batteryTemperature_specify=on  batteryTemperature_priority=High  batteryTemperature=Module09.batteryTemperature K  batteryTemperature_nominal_specify=off  batteryTemperature_nominal_value=1  batteryTemperature_nominal_unit=K  vParallelAssembly_specify=on  vParallelAssembly_priority=None  vParallelAssembly=Module09.vParallelAssembly V  vParallelAssembly_nominal_specify=off  vParallelAssembly_nominal_value=1  vParallelAssembly_nominal_unit=V  socParallelAssembly_specify=on  socParallelAssembly_priority=None  socParallelAssembly=Module09.socParallelAssembly  socParallelAssembly_nominal_specify=off  socParallelAssembly_nominal_value=1  socParallelAssembly_nominal_unit=1
      settings: InternalSimscapePortConfiguration="{\"Bottom\":[{\"id\":\"n\",\"label\":\"-\",\"type\":\"foundation.electrical.electrical\"}],\"Left\":[{\"id\":\"AmbH\",\"label\":\"AmbH\",\"type\":\"foundation.thermal.thermal\"}],\"Right\":[],\"Top\":[{\"id\":\"p\",\"label\":\"+\",\"type\":\"foundation.electrical.electrical\"}]}"
  Module09_outputs : SimscapeProbe  BoundBlock=10  Variables="{\"batteryCurrent\":{\"Probing\":\"ON\"},\"batteryTemperature\":{\"Probing\":\"ON\"},\"batteryVoltage\":{\"Probing\":\"ON\"},\"numCycles\":{\"Probing\":\"ON\"},\"socCell\":{\"Probing\":\"ON\"},\"socParallelAssembly\":{\"Probing\":\"ON\"},\"vParallelAssembly\":{\"Probing\":\"ON\"}}"
  Module10 : thermalCoupledCellResolution_lib/Modules/ModuleType1  BatteryCapacityCell=Module10.BatteryCapacityCell A*hr  BatteryCapacityCellPercentDeviation=Module10.BatteryCapacityCellPercentDeviation  ExtrapolationMethodCell=simscape.enum.extrapolation.nearest  SOCBreakpointsCell=Module10.SOCBreakpointsCell  SOCBreakpointsCellPercentDeviation=Module10.SOCBreakpointsCellPercentDeviation  TemperatureBreakpointsCell=Module10.TemperatureBreakpointsCell K  TemperatureBreakpointsCellPercentDeviation=Module10.TemperatureBreakpointsCellPercentDeviation  OpenCircuitVoltageThermalCell=Module10.OpenCircuitVoltageThermalCell V  OpenCircuitVoltageThermalCellPercentDeviation=Module10.OpenCircuitVoltageThermalCellPercentDeviation  VoltageRangeCell=Module10.VoltageRangeCell V  VoltageRangeCellPercentDeviation=Module10.VoltageRangeCellPercentDeviation  ResistanceSOCBreakpointsCell=Module10.ResistanceSOCBreakpointsCell  ResistanceSOCBreakpointsCellPercentDeviation=Module10.ResistanceSOCBreakpointsCellPercentDeviation  ResistanceTemperatureBreakpointsCell=Module10.ResistanceTemperatureBreakpointsCell K  ResistanceTemperatureBreakpointsCellPercentDeviation=Module10.ResistanceTemperatureBreakpointsCellPercentDeviation  R0ThermalCell=Module10.R0ThermalCell Ohm  R0ThermalCellPercentDeviation=Module10.R0ThermalCellPercentDeviation  R1ThermalCell=Module10.R1ThermalCell Ohm  R1ThermalCellPercentDeviation=Module10.R1ThermalCellPercentDeviation  Tau1ThermalCell=Module10.Tau1ThermalCell s  Tau1ThermalCellPercentDeviation=Module10.Tau1ThermalCellPercentDeviation  BatteryThermalMassCell=Module10.BatteryThermalMassCell J/K  BatteryThermalMassCellPercentDeviation=Module10.BatteryThermalMassCellPercentDeviation  AmbientResistance=Module10.AmbientResistance K/W  P=2  S=6  socCell_specify=on  socCell_priority=High  socCell=Module10.socCell  socCell_nominal_specify=off  socCell_nominal_value=1  socCell_nominal_unit=1  batteryVoltage_specify=on  batteryVoltage_priority=None  batteryVoltage=Module10.batteryVoltage V  batteryVoltage_nominal_specify=off  batteryVoltage_nominal_value=1  batteryVoltage_nominal_unit=V  batteryCurrent_specify=on  batteryCurrent_priority=None  batteryCurrent=Module10.batteryCurrent A  batteryCurrent_nominal_specify=off  batteryCurrent_nominal_value=1  batteryCurrent_nominal_unit=A  numCycles_specify=on  numCycles_priority=High  numCycles=Module10.numCycles  numCycles_nominal_specify=off  numCycles_nominal_value=1  numCycles_nominal_unit=1  batteryTemperature_specify=on  batteryTemperature_priority=High  batteryTemperature=Module10.batteryTemperature K  batteryTemperature_nominal_specify=off  batteryTemperature_nominal_value=1  batteryTemperature_nominal_unit=K  vParallelAssembly_specify=on  vParallelAssembly_priority=None  vParallelAssembly=Module10.vParallelAssembly V  vParallelAssembly_nominal_specify=off  vParallelAssembly_nominal_value=1  vParallelAssembly_nominal_unit=V  socParallelAssembly_specify=on  socParallelAssembly_priority=None  socParallelAssembly=Module10.socParallelAssembly  socParallelAssembly_nominal_specify=off  socParallelAssembly_nominal_value=1  socParallelAssembly_nominal_unit=1
      settings: InternalSimscapePortConfiguration="{\"Bottom\":[{\"id\":\"n\",\"label\":\"-\",\"type\":\"foundation.electrical.electrical\"}],\"Left\":[{\"id\":\"AmbH\",\"label\":\"AmbH\",\"type\":\"foundation.thermal.thermal\"}],\"Right\":[],\"Top\":[{\"id\":\"p\",\"label\":\"+\",\"type\":\"foundation.electrical.electrical\"}]}"
  Module10_outputs : SimscapeProbe  BoundBlock=11  Variables="{\"batteryCurrent\":{\"Probing\":\"ON\"},\"batteryTemperature\":{\"Probing\":\"ON\"},\"batteryVoltage\":{\"Probing\":\"ON\"},\"numCycles\":{\"Probing\":\"ON\"},\"socCell\":{\"Probing\":\"ON\"},\"socParallelAssembly\":{\"Probing\":\"ON\"},\"vParallelAssembly\":{\"Probing\":\"ON\"}}"
  Module11 : thermalCoupledCellResolution_lib/Modules/ModuleType1  BatteryCapacityCell=Module11.BatteryCapacityCell A*hr  BatteryCapacityCellPercentDeviation=Module11.BatteryCapacityCellPercentDeviation  ExtrapolationMethodCell=simscape.enum.extrapolation.nearest  SOCBreakpointsCell=Module11.SOCBreakpointsCell  SOCBreakpointsCellPercentDeviation=Module11.SOCBreakpointsCellPercentDeviation  TemperatureBreakpointsCell=Module11.TemperatureBreakpointsCell K  TemperatureBreakpointsCellPercentDeviation=Module11.TemperatureBreakpointsCellPercentDeviation  OpenCircuitVoltageThermalCell=Module11.OpenCircuitVoltageThermalCell V  OpenCircuitVoltageThermalCellPercentDeviation=Module11.OpenCircuitVoltageThermalCellPercentDeviation  VoltageRangeCell=Module11.VoltageRangeCell V  VoltageRangeCellPercentDeviation=Module11.VoltageRangeCellPercentDeviation  ResistanceSOCBreakpointsCell=Module11.ResistanceSOCBreakpointsCell  ResistanceSOCBreakpointsCellPercentDeviation=Module11.ResistanceSOCBreakpointsCellPercentDeviation  ResistanceTemperatureBreakpointsCell=Module11.ResistanceTemperatureBreakpointsCell K  ResistanceTemperatureBreakpointsCellPercentDeviation=Module11.ResistanceTemperatureBreakpointsCellPercentDeviation  R0ThermalCell=Module11.R0ThermalCell Ohm  R0ThermalCellPercentDeviation=Module11.R0ThermalCellPercentDeviation  R1ThermalCell=Module11.R1ThermalCell Ohm  R1ThermalCellPercentDeviation=Module11.R1ThermalCellPercentDeviation  Tau1ThermalCell=Module11.Tau1ThermalCell s  Tau1ThermalCellPercentDeviation=Module11.Tau1ThermalCellPercentDeviation  BatteryThermalMassCell=Module11.BatteryThermalMassCell J/K  BatteryThermalMassCellPercentDeviation=Module11.BatteryThermalMassCellPercentDeviation  AmbientResistance=Module11.AmbientResistance K/W  P=2  S=6  socCell_specify=on  socCell_priority=High  socCell=Module11.socCell  socCell_nominal_specify=off  socCell_nominal_value=1  socCell_nominal_unit=1  batteryVoltage_specify=on  batteryVoltage_priority=None  batteryVoltage=Module11.batteryVoltage V  batteryVoltage_nominal_specify=off  batteryVoltage_nominal_value=1  batteryVoltage_nominal_unit=V  batteryCurrent_specify=on  batteryCurrent_priority=None  batteryCurrent=Module11.batteryCurrent A  batteryCurrent_nominal_specify=off  batteryCurrent_nominal_value=1  batteryCurrent_nominal_unit=A  numCycles_specify=on  numCycles_priority=High  numCycles=Module11.numCycles  numCycles_nominal_specify=off  numCycles_nominal_value=1  numCycles_nominal_unit=1  batteryTemperature_specify=on  batteryTemperature_priority=High  batteryTemperature=Module11.batteryTemperature K  batteryTemperature_nominal_specify=off  batteryTemperature_nominal_value=1  batteryTemperature_nominal_unit=K  vParallelAssembly_specify=on  vParallelAssembly_priority=None  vParallelAssembly=Module11.vParallelAssembly V  vParallelAssembly_nominal_specify=off  vParallelAssembly_nominal_value=1  vParallelAssembly_nominal_unit=V  socParallelAssembly_specify=on  socParallelAssembly_priority=None  socParallelAssembly=Module11.socParallelAssembly  socParallelAssembly_nominal_specify=off  socParallelAssembly_nominal_value=1  socParallelAssembly_nominal_unit=1
      settings: InternalSimscapePortConfiguration="{\"Bottom\":[{\"id\":\"n\",\"label\":\"-\",\"type\":\"foundation.electrical.electrical\"}],\"Left\":[{\"id\":\"AmbH\",\"label\":\"AmbH\",\"type\":\"foundation.thermal.thermal\"}],\"Right\":[],\"Top\":[{\"id\":\"p\",\"label\":\"+\",\"type\":\"foundation.electrical.electrical\"}]}"
  Module11_outputs : SimscapeProbe  BoundBlock=12  Variables="{\"batteryCurrent\":{\"Probing\":\"ON\"},\"batteryTemperature\":{\"Probing\":\"ON\"},\"batteryVoltage\":{\"Probing\":\"ON\"},\"numCycles\":{\"Probing\":\"ON\"},\"socCell\":{\"Probing\":\"ON\"},\"socParallelAssembly\":{\"Probing\":\"ON\"},\"vParallelAssembly\":{\"Probing\":\"ON\"}}"
  Module12 : thermalCoupledCellResolution_lib/Modules/ModuleType1  BatteryCapacityCell=Module12.BatteryCapacityCell A*hr  BatteryCapacityCellPercentDeviation=Module12.BatteryCapacityCellPercentDeviation  ExtrapolationMethodCell=simscape.enum.extrapolation.nearest  SOCBreakpointsCell=Module12.SOCBreakpointsCell  SOCBreakpointsCellPercentDeviation=Module12.SOCBreakpointsCellPercentDeviation  TemperatureBreakpointsCell=Module12.TemperatureBreakpointsCell K  TemperatureBreakpointsCellPercentDeviation=Module12.TemperatureBreakpointsCellPercentDeviation  OpenCircuitVoltageThermalCell=Module12.OpenCircuitVoltageThermalCell V  OpenCircuitVoltageThermalCellPercentDeviation=Module12.OpenCircuitVoltageThermalCellPercentDeviation  VoltageRangeCell=Module12.VoltageRangeCell V  VoltageRangeCellPercentDeviation=Module12.VoltageRangeCellPercentDeviation  ResistanceSOCBreakpointsCell=Module12.ResistanceSOCBreakpointsCell  ResistanceSOCBreakpointsCellPercentDeviation=Module12.ResistanceSOCBreakpointsCellPercentDeviation  ResistanceTemperatureBreakpointsCell=Module12.ResistanceTemperatureBreakpointsCell K  ResistanceTemperatureBreakpointsCellPercentDeviation=Module12.ResistanceTemperatureBreakpointsCellPercentDeviation  R0ThermalCell=Module12.R0ThermalCell Ohm  R0ThermalCellPercentDeviation=Module12.R0ThermalCellPercentDeviation  R1ThermalCell=Module12.R1ThermalCell Ohm  R1ThermalCellPercentDeviation=Module12.R1ThermalCellPercentDeviation  Tau1ThermalCell=Module12.Tau1ThermalCell s  Tau1ThermalCellPercentDeviation=Module12.Tau1ThermalCellPercentDeviation  BatteryThermalMassCell=Module12.BatteryThermalMassCell J/K  BatteryThermalMassCellPercentDeviation=Module12.BatteryThermalMassCellPercentDeviation  AmbientResistance=Module12.AmbientResistance K/W  P=2  S=6  socCell_specify=on  socCell_priority=High  socCell=Module12.socCell  socCell_nominal_specify=off  socCell_nominal_value=1  socCell_nominal_unit=1  batteryVoltage_specify=on  batteryVoltage_priority=None  batteryVoltage=Module12.batteryVoltage V  batteryVoltage_nominal_specify=off  batteryVoltage_nominal_value=1  batteryVoltage_nominal_unit=V  batteryCurrent_specify=on  batteryCurrent_priority=None  batteryCurrent=Module12.batteryCurrent A  batteryCurrent_nominal_specify=off  batteryCurrent_nominal_value=1  batteryCurrent_nominal_unit=A  numCycles_specify=on  numCycles_priority=High  numCycles=Module12.numCycles  numCycles_nominal_specify=off  numCycles_nominal_value=1  numCycles_nominal_unit=1  batteryTemperature_specify=on  batteryTemperature_priority=High  batteryTemperature=Module12.batteryTemperature K  batteryTemperature_nominal_specify=off  batteryTemperature_nominal_value=1  batteryTemperature_nominal_unit=K  vParallelAssembly_specify=on  vParallelAssembly_priority=None  vParallelAssembly=Module12.vParallelAssembly V  vParallelAssembly_nominal_specify=off  vParallelAssembly_nominal_value=1  vParallelAssembly_nominal_unit=V  socParallelAssembly_specify=on  socParallelAssembly_priority=None  socParallelAssembly=Module12.socParallelAssembly  socParallelAssembly_nominal_specify=off  socParallelAssembly_nominal_value=1  socParallelAssembly_nominal_unit=1
      settings: InternalSimscapePortConfiguration="{\"Bottom\":[{\"id\":\"n\",\"label\":\"-\",\"type\":\"foundation.electrical.electrical\"}],\"Left\":[{\"id\":\"AmbH\",\"label\":\"AmbH\",\"type\":\"foundation.thermal.thermal\"}],\"Right\":[],\"Top\":[{\"id\":\"p\",\"label\":\"+\",\"type\":\"foundation.electrical.electrical\"}]}"
  Module12_outputs : SimscapeProbe  BoundBlock=13  Variables="{\"batteryCurrent\":{\"Probing\":\"ON\"},\"batteryTemperature\":{\"Probing\":\"ON\"},\"batteryVoltage\":{\"Probing\":\"ON\"},\"numCycles\":{\"Probing\":\"ON\"},\"socCell\":{\"Probing\":\"ON\"},\"socParallelAssembly\":{\"Probing\":\"ON\"},\"vParallelAssembly\":{\"Probing\":\"ON\"}}"
  Module13 : thermalCoupledCellResolution_lib/Modules/ModuleType1  BatteryCapacityCell=Module13.BatteryCapacityCell A*hr  BatteryCapacityCellPercentDeviation=Module13.BatteryCapacityCellPercentDeviation  ExtrapolationMethodCell=simscape.enum.extrapolation.nearest  SOCBreakpointsCell=Module13.SOCBreakpointsCell  SOCBreakpointsCellPercentDeviation=Module13.SOCBreakpointsCellPercentDeviation  TemperatureBreakpointsCell=Module13.TemperatureBreakpointsCell K  TemperatureBreakpointsCellPercentDeviation=Module13.TemperatureBreakpointsCellPercentDeviation  OpenCircuitVoltageThermalCell=Module13.OpenCircuitVoltageThermalCell V  OpenCircuitVoltageThermalCellPercentDeviation=Module13.OpenCircuitVoltageThermalCellPercentDeviation  VoltageRangeCell=Module13.VoltageRangeCell V  VoltageRangeCellPercentDeviation=Module13.VoltageRangeCellPercentDeviation  ResistanceSOCBreakpointsCell=Module13.ResistanceSOCBreakpointsCell  ResistanceSOCBreakpointsCellPercentDeviation=Module13.ResistanceSOCBreakpointsCellPercentDeviation  ResistanceTemperatureBreakpointsCell=Module13.ResistanceTemperatureBreakpointsCell K  ResistanceTemperatureBreakpointsCellPercentDeviation=Module13.ResistanceTemperatureBreakpointsCellPercentDeviation  R0ThermalCell=Module13.R0ThermalCell Ohm  R0ThermalCellPercentDeviation=Module13.R0ThermalCellPercentDeviation  R1ThermalCell=Module13.R1ThermalCell Ohm  R1ThermalCellPercentDeviation=Module13.R1ThermalCellPercentDeviation  Tau1ThermalCell=Module13.Tau1ThermalCell s  Tau1ThermalCellPercentDeviation=Module13.Tau1ThermalCellPercentDeviation  BatteryThermalMassCell=Module13.BatteryThermalMassCell J/K  BatteryThermalMassCellPercentDeviation=Module13.BatteryThermalMassCellPercentDeviation  AmbientResistance=Module13.AmbientResistance K/W  P=2  S=6  socCell_specify=on  socCell_priority=High  socCell=Module13.socCell  socCell_nominal_specify=off  socCell_nominal_value=1  socCell_nominal_unit=1  batteryVoltage_specify=on  batteryVoltage_priority=None  batteryVoltage=Module13.batteryVoltage V  batteryVoltage_nominal_specify=off  batteryVoltage_nominal_value=1  batteryVoltage_nominal_unit=V  batteryCurrent_specify=on  batteryCurrent_priority=None  batteryCurrent=Module13.batteryCurrent A  batteryCurrent_nominal_specify=off  batteryCurrent_nominal_value=1  batteryCurrent_nominal_unit=A  numCycles_specify=on  numCycles_priority=High  numCycles=Module13.numCycles  numCycles_nominal_specify=off  numCycles_nominal_value=1  numCycles_nominal_unit=1  batteryTemperature_specify=on  batteryTemperature_priority=High  batteryTemperature=Module13.batteryTemperature K  batteryTemperature_nominal_specify=off  batteryTemperature_nominal_value=1  batteryTemperature_nominal_unit=K  vParallelAssembly_specify=on  vParallelAssembly_priority=None  vParallelAssembly=Module13.vParallelAssembly V  vParallelAssembly_nominal_specify=off  vParallelAssembly_nominal_value=1  vParallelAssembly_nominal_unit=V  socParallelAssembly_specify=on  socParallelAssembly_priority=None  socParallelAssembly=Module13.socParallelAssembly  socParallelAssembly_nominal_specify=off  socParallelAssembly_nominal_value=1  socParallelAssembly_nominal_unit=1
      settings: InternalSimscapePortConfiguration="{\"Bottom\":[{\"id\":\"n\",\"label\":\"-\",\"type\":\"foundation.electrical.electrical\"}],\"Left\":[{\"id\":\"AmbH\",\"label\":\"AmbH\",\"type\":\"foundation.thermal.thermal\"}],\"Right\":[],\"Top\":[{\"id\":\"p\",\"label\":\"+\",\"type\":\"foundation.electrical.electrical\"}]}"
  Module13_outputs : SimscapeProbe  BoundBlock=14  Variables="{\"batteryCurrent\":{\"Probing\":\"ON\"},\"batteryTemperature\":{\"Probing\":\"ON\"},\"batteryVoltage\":{\"Probing\":\"ON\"},\"numCycles\":{\"Probing\":\"ON\"},\"socCell\":{\"Probing\":\"ON\"},\"socParallelAssembly\":{\"Probing\":\"ON\"},\"vParallelAssembly\":{\"Probing\":\"ON\"}}"
  Module14 : thermalCoupledCellResolution_lib/Modules/ModuleType1  BatteryCapacityCell=Module14.BatteryCapacityCell A*hr  BatteryCapacityCellPercentDeviation=Module14.BatteryCapacityCellPercentDeviation  ExtrapolationMethodCell=simscape.enum.extrapolation.nearest  SOCBreakpointsCell=Module14.SOCBreakpointsCell  SOCBreakpointsCellPercentDeviation=Module14.SOCBreakpointsCellPercentDeviation  TemperatureBreakpointsCell=Module14.TemperatureBreakpointsCell K  TemperatureBreakpointsCellPercentDeviation=Module14.TemperatureBreakpointsCellPercentDeviation  OpenCircuitVoltageThermalCell=Module14.OpenCircuitVoltageThermalCell V  OpenCircuitVoltageThermalCellPercentDeviation=Module14.OpenCircuitVoltageThermalCellPercentDeviation  VoltageRangeCell=Module14.VoltageRangeCell V  VoltageRangeCellPercentDeviation=Module14.VoltageRangeCellPercentDeviation  ResistanceSOCBreakpointsCell=Module14.ResistanceSOCBreakpointsCell  ResistanceSOCBreakpointsCellPercentDeviation=Module14.ResistanceSOCBreakpointsCellPercentDeviation  ResistanceTemperatureBreakpointsCell=Module14.ResistanceTemperatureBreakpointsCell K  ResistanceTemperatureBreakpointsCellPercentDeviation=Module14.ResistanceTemperatureBreakpointsCellPercentDeviation  R0ThermalCell=Module14.R0ThermalCell Ohm  R0ThermalCellPercentDeviation=Module14.R0ThermalCellPercentDeviation  R1ThermalCell=Module14.R1ThermalCell Ohm  R1ThermalCellPercentDeviation=Module14.R1ThermalCellPercentDeviation  Tau1ThermalCell=Module14.Tau1ThermalCell s  Tau1ThermalCellPercentDeviation=Module14.Tau1ThermalCellPercentDeviation  BatteryThermalMassCell=Module14.BatteryThermalMassCell J/K  BatteryThermalMassCellPercentDeviation=Module14.BatteryThermalMassCellPercentDeviation  AmbientResistance=Module14.AmbientResistance K/W  P=2  S=6  socCell_specify=on  socCell_priority=High  socCell=Module14.socCell  socCell_nominal_specify=off  socCell_nominal_value=1  socCell_nominal_unit=1  batteryVoltage_specify=on  batteryVoltage_priority=None  batteryVoltage=Module14.batteryVoltage V  batteryVoltage_nominal_specify=off  batteryVoltage_nominal_value=1  batteryVoltage_nominal_unit=V  batteryCurrent_specify=on  batteryCurrent_priority=None  batteryCurrent=Module14.batteryCurrent A  batteryCurrent_nominal_specify=off  batteryCurrent_nominal_value=1  batteryCurrent_nominal_unit=A  numCycles_specify=on  numCycles_priority=High  numCycles=Module14.numCycles  numCycles_nominal_specify=off  numCycles_nominal_value=1  numCycles_nominal_unit=1  batteryTemperature_specify=on  batteryTemperature_priority=High  batteryTemperature=Module14.batteryTemperature K  batteryTemperature_nominal_specify=off  batteryTemperature_nominal_value=1  batteryTemperature_nominal_unit=K  vParallelAssembly_specify=on  vParallelAssembly_priority=None  vParallelAssembly=Module14.vParallelAssembly V  vParallelAssembly_nominal_specify=off  vParallelAssembly_nominal_value=1  vParallelAssembly_nominal_unit=V  socParallelAssembly_specify=on  socParallelAssembly_priority=None  socParallelAssembly=Module14.socParallelAssembly  socParallelAssembly_nominal_specify=off  socParallelAssembly_nominal_value=1  socParallelAssembly_nominal_unit=1
      settings: InternalSimscapePortConfiguration="{\"Bottom\":[{\"id\":\"n\",\"label\":\"-\",\"type\":\"foundation.electrical.electrical\"}],\"Left\":[{\"id\":\"AmbH\",\"label\":\"AmbH\",\"type\":\"foundation.thermal.thermal\"}],\"Right\":[],\"Top\":[{\"id\":\"p\",\"label\":\"+\",\"type\":\"foundation.electrical.electrical\"}]}"
  Module14_outputs : SimscapeProbe  BoundBlock=15  Variables="{\"batteryCurrent\":{\"Probing\":\"ON\"},\"batteryTemperature\":{\"Probing\":\"ON\"},\"batteryVoltage\":{\"Probing\":\"ON\"},\"numCycles\":{\"Probing\":\"ON\"},\"socCell\":{\"Probing\":\"ON\"},\"socParallelAssembly\":{\"Probing\":\"ON\"},\"vParallelAssembly\":{\"Probing\":\"ON\"}}"
  Module15 : thermalCoupledCellResolution_lib/Modules/ModuleType1  BatteryCapacityCell=Module15.BatteryCapacityCell A*hr  BatteryCapacityCellPercentDeviation=Module15.BatteryCapacityCellPercentDeviation  ExtrapolationMethodCell=simscape.enum.extrapolation.nearest  SOCBreakpointsCell=Module15.SOCBreakpointsCell  SOCBreakpointsCellPercentDeviation=Module15.SOCBreakpointsCellPercentDeviation  TemperatureBreakpointsCell=Module15.TemperatureBreakpointsCell K  TemperatureBreakpointsCellPercentDeviation=Module15.TemperatureBreakpointsCellPercentDeviation  OpenCircuitVoltageThermalCell=Module15.OpenCircuitVoltageThermalCell V  OpenCircuitVoltageThermalCellPercentDeviation=Module15.OpenCircuitVoltageThermalCellPercentDeviation  VoltageRangeCell=Module15.VoltageRangeCell V  VoltageRangeCellPercentDeviation=Module15.VoltageRangeCellPercentDeviation  ResistanceSOCBreakpointsCell=Module15.ResistanceSOCBreakpointsCell  ResistanceSOCBreakpointsCellPercentDeviation=Module15.ResistanceSOCBreakpointsCellPercentDeviation  ResistanceTemperatureBreakpointsCell=Module15.ResistanceTemperatureBreakpointsCell K  ResistanceTemperatureBreakpointsCellPercentDeviation=Module15.ResistanceTemperatureBreakpointsCellPercentDeviation  R0ThermalCell=Module15.R0ThermalCell Ohm  R0ThermalCellPercentDeviation=Module15.R0ThermalCellPercentDeviation  R1ThermalCell=Module15.R1ThermalCell Ohm  R1ThermalCellPercentDeviation=Module15.R1ThermalCellPercentDeviation  Tau1ThermalCell=Module15.Tau1ThermalCell s  Tau1ThermalCellPercentDeviation=Module15.Tau1ThermalCellPercentDeviation  BatteryThermalMassCell=Module15.BatteryThermalMassCell J/K  BatteryThermalMassCellPercentDeviation=Module15.BatteryThermalMassCellPercentDeviation  AmbientResistance=Module15.AmbientResistance K/W  P=2  S=6  socCell_specify=on  socCell_priority=High  socCell=Module15.socCell  socCell_nominal_specify=off  socCell_nominal_value=1  socCell_nominal_unit=1  batteryVoltage_specify=on  batteryVoltage_priority=None  batteryVoltage=Module15.batteryVoltage V  batteryVoltage_nominal_specify=off  batteryVoltage_nominal_value=1  batteryVoltage_nominal_unit=V  batteryCurrent_specify=on  batteryCurrent_priority=None  batteryCurrent=Module15.batteryCurrent A  batteryCurrent_nominal_specify=off  batteryCurrent_nominal_value=1  batteryCurrent_nominal_unit=A  numCycles_specify=on  numCycles_priority=High  numCycles=Module15.numCycles  numCycles_nominal_specify=off  numCycles_nominal_value=1  numCycles_nominal_unit=1  batteryTemperature_specify=on  batteryTemperature_priority=High  batteryTemperature=Module15.batteryTemperature K  batteryTemperature_nominal_specify=off  batteryTemperature_nominal_value=1  batteryTemperature_nominal_unit=K  vParallelAssembly_specify=on  vParallelAssembly_priority=None  vParallelAssembly=Module15.vParallelAssembly V  vParallelAssembly_nominal_specify=off  vParallelAssembly_nominal_value=1  vParallelAssembly_nominal_unit=V  socParallelAssembly_specify=on  socParallelAssembly_priority=None  socParallelAssembly=Module15.socParallelAssembly  socParallelAssembly_nominal_specify=off  socParallelAssembly_nominal_value=1  socParallelAssembly_nominal_unit=1
      settings: InternalSimscapePortConfiguration="{\"Bottom\":[{\"id\":\"n\",\"label\":\"-\",\"type\":\"foundation.electrical.electrical\"}],\"Left\":[{\"id\":\"AmbH\",\"label\":\"AmbH\",\"type\":\"foundation.thermal.thermal\"}],\"Right\":[],\"Top\":[{\"id\":\"p\",\"label\":\"+\",\"type\":\"foundation.electrical.electrical\"}]}"
  Module15_outputs : SimscapeProbe  BoundBlock=16  Variables="{\"batteryCurrent\":{\"Probing\":\"ON\"},\"batteryTemperature\":{\"Probing\":\"ON\"},\"batteryVoltage\":{\"Probing\":\"ON\"},\"numCycles\":{\"Probing\":\"ON\"},\"socCell\":{\"Probing\":\"ON\"},\"socParallelAssembly\":{\"Probing\":\"ON\"},\"vParallelAssembly\":{\"Probing\":\"ON\"}}"
  Module16 : thermalCoupledCellResolution_lib/Modules/ModuleType1  BatteryCapacityCell=Module16.BatteryCapacityCell A*hr  BatteryCapacityCellPercentDeviation=Module16.BatteryCapacityCellPercentDeviation  ExtrapolationMethodCell=simscape.enum.extrapolation.nearest  SOCBreakpointsCell=Module16.SOCBreakpointsCell  SOCBreakpointsCellPercentDeviation=Module16.SOCBreakpointsCellPercentDeviation  TemperatureBreakpointsCell=Module16.TemperatureBreakpointsCell K  TemperatureBreakpointsCellPercentDeviation=Module16.TemperatureBreakpointsCellPercentDeviation  OpenCircuitVoltageThermalCell=Module16.OpenCircuitVoltageThermalCell V  OpenCircuitVoltageThermalCellPercentDeviation=Module16.OpenCircuitVoltageThermalCellPercentDeviation  VoltageRangeCell=Module16.VoltageRangeCell V  VoltageRangeCellPercentDeviation=Module16.VoltageRangeCellPercentDeviation  ResistanceSOCBreakpointsCell=Module16.ResistanceSOCBreakpointsCell  ResistanceSOCBreakpointsCellPercentDeviation=Module16.ResistanceSOCBreakpointsCellPercentDeviation  ResistanceTemperatureBreakpointsCell=Module16.ResistanceTemperatureBreakpointsCell K  ResistanceTemperatureBreakpointsCellPercentDeviation=Module16.ResistanceTemperatureBreakpointsCellPercentDeviation  R0ThermalCell=Module16.R0ThermalCell Ohm  R0ThermalCellPercentDeviation=Module16.R0ThermalCellPercentDeviation  R1ThermalCell=Module16.R1ThermalCell Ohm  R1ThermalCellPercentDeviation=Module16.R1ThermalCellPercentDeviation  Tau1ThermalCell=Module16.Tau1ThermalCell s  Tau1ThermalCellPercentDeviation=Module16.Tau1ThermalCellPercentDeviation  BatteryThermalMassCell=Module16.BatteryThermalMassCell J/K  BatteryThermalMassCellPercentDeviation=Module16.BatteryThermalMassCellPercentDeviation  AmbientResistance=Module16.AmbientResistance K/W  P=2  S=6  socCell_specify=on  socCell_priority=High  socCell=Module16.socCell  socCell_nominal_specify=off  socCell_nominal_value=1  socCell_nominal_unit=1  batteryVoltage_specify=on  batteryVoltage_priority=None  batteryVoltage=Module16.batteryVoltage V  batteryVoltage_nominal_specify=off  batteryVoltage_nominal_value=1  batteryVoltage_nominal_unit=V  batteryCurrent_specify=on  batteryCurrent_priority=None  batteryCurrent=Module16.batteryCurrent A  batteryCurrent_nominal_specify=off  batteryCurrent_nominal_value=1  batteryCurrent_nominal_unit=A  numCycles_specify=on  numCycles_priority=High  numCycles=Module16.numCycles  numCycles_nominal_specify=off  numCycles_nominal_value=1  numCycles_nominal_unit=1  batteryTemperature_specify=on  batteryTemperature_priority=High  batteryTemperature=Module16.batteryTemperature K  batteryTemperature_nominal_specify=off  batteryTemperature_nominal_value=1  batteryTemperature_nominal_unit=K  vParallelAssembly_specify=on  vParallelAssembly_priority=None  vParallelAssembly=Module16.vParallelAssembly V  vParallelAssembly_nominal_specify=off  vParallelAssembly_nominal_value=1  vParallelAssembly_nominal_unit=V  socParallelAssembly_specify=on  socParallelAssembly_priority=None  socParallelAssembly=Module16.socParallelAssembly  socParallelAssembly_nominal_specify=off  socParallelAssembly_nominal_value=1  socParallelAssembly_nominal_unit=1
      settings: InternalSimscapePortConfiguration="{\"Bottom\":[{\"id\":\"n\",\"label\":\"-\",\"type\":\"foundation.electrical.electrical\"}],\"Left\":[{\"id\":\"AmbH\",\"label\":\"AmbH\",\"type\":\"foundation.thermal.thermal\"}],\"Right\":[],\"Top\":[{\"id\":\"p\",\"label\":\"+\",\"type\":\"foundation.electrical.electrical\"}]}"
  Module16_outputs : SimscapeProbe  BoundBlock=17  Variables="{\"batteryCurrent\":{\"Probing\":\"ON\"},\"batteryTemperature\":{\"Probing\":\"ON\"},\"batteryVoltage\":{\"Probing\":\"ON\"},\"numCycles\":{\"Probing\":\"ON\"},\"socCell\":{\"Probing\":\"ON\"},\"socParallelAssembly\":{\"Probing\":\"ON\"},\"vParallelAssembly\":{\"Probing\":\"ON\"}}"
  Module17 : thermalCoupledCellResolution_lib/Modules/ModuleType1  BatteryCapacityCell=Module17.BatteryCapacityCell A*hr  BatteryCapacityCellPercentDeviation=Module17.BatteryCapacityCellPercentDeviation  ExtrapolationMethodCell=simscape.enum.extrapolation.nearest  SOCBreakpointsCell=Module17.SOCBreakpointsCell  SOCBreakpointsCellPercentDeviation=Module17.SOCBreakpointsCellPercentDeviation  TemperatureBreakpointsCell=Module17.TemperatureBreakpointsCell K  TemperatureBreakpointsCellPercentDeviation=Module17.TemperatureBreakpointsCellPercentDeviation  OpenCircuitVoltageThermalCell=Module17.OpenCircuitVoltageThermalCell V  OpenCircuitVoltageThermalCellPercentDeviation=Module17.OpenCircuitVoltageThermalCellPercentDeviation  VoltageRangeCell=Module17.VoltageRangeCell V  VoltageRangeCellPercentDeviation=Module17.VoltageRangeCellPercentDeviation  ResistanceSOCBreakpointsCell=Module17.ResistanceSOCBreakpointsCell  ResistanceSOCBreakpointsCellPercentDeviation=Module17.ResistanceSOCBreakpointsCellPercentDeviation  ResistanceTemperatureBreakpointsCell=Module17.ResistanceTemperatureBreakpointsCell K  ResistanceTemperatureBreakpointsCellPercentDeviation=Module17.ResistanceTemperatureBreakpointsCellPercentDeviation  R0ThermalCell=Module17.R0ThermalCell Ohm  R0ThermalCellPercentDeviation=Module17.R0ThermalCellPercentDeviation  R1ThermalCell=Module17.R1ThermalCell Ohm  R1ThermalCellPercentDeviation=Module17.R1ThermalCellPercentDeviation  Tau1ThermalCell=Module17.Tau1ThermalCell s  Tau1ThermalCellPercentDeviation=Module17.Tau1ThermalCellPercentDeviation  BatteryThermalMassCell=Module17.BatteryThermalMassCell J/K  BatteryThermalMassCellPercentDeviation=Module17.BatteryThermalMassCellPercentDeviation  AmbientResistance=Module17.AmbientResistance K/W  P=2  S=6  socCell_specify=on  socCell_priority=High  socCell=Module17.socCell  socCell_nominal_specify=off  socCell_nominal_value=1  socCell_nominal_unit=1  batteryVoltage_specify=on  batteryVoltage_priority=None  batteryVoltage=Module17.batteryVoltage V  batteryVoltage_nominal_specify=off  batteryVoltage_nominal_value=1  batteryVoltage_nominal_unit=V  batteryCurrent_specify=on  batteryCurrent_priority=None  batteryCurrent=Module17.batteryCurrent A  batteryCurrent_nominal_specify=off  batteryCurrent_nominal_value=1  batteryCurrent_nominal_unit=A  numCycles_specify=on  numCycles_priority=High  numCycles=Module17.numCycles  numCycles_nominal_specify=off  numCycles_nominal_value=1  numCycles_nominal_unit=1  batteryTemperature_specify=on  batteryTemperature_priority=High  batteryTemperature=Module17.batteryTemperature K  batteryTemperature_nominal_specify=off  batteryTemperature_nominal_value=1  batteryTemperature_nominal_unit=K  vParallelAssembly_specify=on  vParallelAssembly_priority=None  vParallelAssembly=Module17.vParallelAssembly V  vParallelAssembly_nominal_specify=off  vParallelAssembly_nominal_value=1  vParallelAssembly_nominal_unit=V  socParallelAssembly_specify=on  socParallelAssembly_priority=None  socParallelAssembly=Module17.socParallelAssembly  socParallelAssembly_nominal_specify=off  socParallelAssembly_nominal_value=1  socParallelAssembly_nominal_unit=1
      settings: InternalSimscapePortConfiguration="{\"Bottom\":[{\"id\":\"n\",\"label\":\"-\",\"type\":\"foundation.electrical.electrical\"}],\"Left\":[{\"id\":\"AmbH\",\"label\":\"AmbH\",\"type\":\"foundation.thermal.thermal\"}],\"Right\":[],\"Top\":[{\"id\":\"p\",\"label\":\"+\",\"type\":\"foundation.electrical.electrical\"}]}"
  Module17_outputs : SimscapeProbe  BoundBlock=18  Variables="{\"batteryCurrent\":{\"Probing\":\"ON\"},\"batteryTemperature\":{\"Probing\":\"ON\"},\"batteryVoltage\":{\"Probing\":\"ON\"},\"numCycles\":{\"Probing\":\"ON\"},\"socCell\":{\"Probing\":\"ON\"},\"socParallelAssembly\":{\"Probing\":\"ON\"},\"vParallelAssembly\":{\"Probing\":\"ON\"}}"
  Module18 : thermalCoupledCellResolution_lib/Modules/ModuleType1  BatteryCapacityCell=Module18.BatteryCapacityCell A*hr  BatteryCapacityCellPercentDeviation=Module18.BatteryCapacityCellPercentDeviation  ExtrapolationMethodCell=simscape.enum.extrapolation.nearest  SOCBreakpointsCell=Module18.SOCBreakpointsCell  SOCBreakpointsCellPercentDeviation=Module18.SOCBreakpointsCellPercentDeviation  TemperatureBreakpointsCell=Module18.TemperatureBreakpointsCell K  TemperatureBreakpointsCellPercentDeviation=Module18.TemperatureBreakpointsCellPercentDeviation  OpenCircuitVoltageThermalCell=Module18.OpenCircuitVoltageThermalCell V  OpenCircuitVoltageThermalCellPercentDeviation=Module18.OpenCircuitVoltageThermalCellPercentDeviation  VoltageRangeCell=Module18.VoltageRangeCell V  VoltageRangeCellPercentDeviation=Module18.VoltageRangeCellPercentDeviation  ResistanceSOCBreakpointsCell=Module18.ResistanceSOCBreakpointsCell  ResistanceSOCBreakpointsCellPercentDeviation=Module18.ResistanceSOCBreakpointsCellPercentDeviation  ResistanceTemperatureBreakpointsCell=Module18.ResistanceTemperatureBreakpointsCell K  ResistanceTemperatureBreakpointsCellPercentDeviation=Module18.ResistanceTemperatureBreakpointsCellPercentDeviation  R0ThermalCell=Module18.R0ThermalCell Ohm  R0ThermalCellPercentDeviation=Module18.R0ThermalCellPercentDeviation  R1ThermalCell=Module18.R1ThermalCell Ohm  R1ThermalCellPercentDeviation=Module18.R1ThermalCellPercentDeviation  Tau1ThermalCell=Module18.Tau1ThermalCell s  Tau1ThermalCellPercentDeviation=Module18.Tau1ThermalCellPercentDeviation  BatteryThermalMassCell=Module18.BatteryThermalMassCell J/K  BatteryThermalMassCellPercentDeviation=Module18.BatteryThermalMassCellPercentDeviation  AmbientResistance=Module18.AmbientResistance K/W  P=2  S=6  socCell_specify=on  socCell_priority=High  socCell=Module18.socCell  socCell_nominal_specify=off  socCell_nominal_value=1  socCell_nominal_unit=1  batteryVoltage_specify=on  batteryVoltage_priority=None  batteryVoltage=Module18.batteryVoltage V  batteryVoltage_nominal_specify=off  batteryVoltage_nominal_value=1  batteryVoltage_nominal_unit=V  batteryCurrent_specify=on  batteryCurrent_priority=None  batteryCurrent=Module18.batteryCurrent A  batteryCurrent_nominal_specify=off  batteryCurrent_nominal_value=1  batteryCurrent_nominal_unit=A  numCycles_specify=on  numCycles_priority=High  numCycles=Module18.numCycles  numCycles_nominal_specify=off  numCycles_nominal_value=1  numCycles_nominal_unit=1  batteryTemperature_specify=on  batteryTemperature_priority=High  batteryTemperature=Module18.batteryTemperature K  batteryTemperature_nominal_specify=off  batteryTemperature_nominal_value=1  batteryTemperature_nominal_unit=K  vParallelAssembly_specify=on  vParallelAssembly_priority=None  vParallelAssembly=Module18.vParallelAssembly V  vParallelAssembly_nominal_specify=off  vParallelAssembly_nominal_value=1  vParallelAssembly_nominal_unit=V  socParallelAssembly_specify=on  socParallelAssembly_priority=None  socParallelAssembly=Module18.socParallelAssembly  socParallelAssembly_nominal_specify=off  socParallelAssembly_nominal_value=1  socParallelAssembly_nominal_unit=1
      settings: InternalSimscapePortConfiguration="{\"Bottom\":[{\"id\":\"n\",\"label\":\"-\",\"type\":\"foundation.electrical.electrical\"}],\"Left\":[{\"id\":\"AmbH\",\"label\":\"AmbH\",\"type\":\"foundation.thermal.thermal\"}],\"Right\":[],\"Top\":[{\"id\":\"p\",\"label\":\"+\",\"type\":\"foundation.electrical.electrical\"}]}"
  Module18_outputs : SimscapeProbe  BoundBlock=19  Variables="{\"batteryCurrent\":{\"Probing\":\"ON\"},\"batteryTemperature\":{\"Probing\":\"ON\"},\"batteryVoltage\":{\"Probing\":\"ON\"},\"numCycles\":{\"Probing\":\"ON\"},\"socCell\":{\"Probing\":\"ON\"},\"socParallelAssembly\":{\"Probing\":\"ON\"},\"vParallelAssembly\":{\"Probing\":\"ON\"}}"
  Module19 : thermalCoupledCellResolution_lib/Modules/ModuleType1  BatteryCapacityCell=Module19.BatteryCapacityCell A*hr  BatteryCapacityCellPercentDeviation=Module19.BatteryCapacityCellPercentDeviation  ExtrapolationMethodCell=simscape.enum.extrapolation.nearest  SOCBreakpointsCell=Module19.SOCBreakpointsCell  SOCBreakpointsCellPercentDeviation=Module19.SOCBreakpointsCellPercentDeviation  TemperatureBreakpointsCell=Module19.TemperatureBreakpointsCell K  TemperatureBreakpointsCellPercentDeviation=Module19.TemperatureBreakpointsCellPercentDeviation  OpenCircuitVoltageThermalCell=Module19.OpenCircuitVoltageThermalCell V  OpenCircuitVoltageThermalCellPercentDeviation=Module19.OpenCircuitVoltageThermalCellPercentDeviation  VoltageRangeCell=Module19.VoltageRangeCell V  VoltageRangeCellPercentDeviation=Module19.VoltageRangeCellPercentDeviation  ResistanceSOCBreakpointsCell=Module19.ResistanceSOCBreakpointsCell  ResistanceSOCBreakpointsCellPercentDeviation=Module19.ResistanceSOCBreakpointsCellPercentDeviation  ResistanceTemperatureBreakpointsCell=Module19.ResistanceTemperatureBreakpointsCell K  ResistanceTemperatureBreakpointsCellPercentDeviation=Module19.ResistanceTemperatureBreakpointsCellPercentDeviation  R0ThermalCell=Module19.R0ThermalCell Ohm  R0ThermalCellPercentDeviation=Module19.R0ThermalCellPercentDeviation  R1ThermalCell=Module19.R1ThermalCell Ohm  R1ThermalCellPercentDeviation=Module19.R1ThermalCellPercentDeviation  Tau1ThermalCell=Module19.Tau1ThermalCell s  Tau1ThermalCellPercentDeviation=Module19.Tau1ThermalCellPercentDeviation  BatteryThermalMassCell=Module19.BatteryThermalMassCell J/K  BatteryThermalMassCellPercentDeviation=Module19.BatteryThermalMassCellPercentDeviation  AmbientResistance=Module19.AmbientResistance K/W  P=2  S=6  socCell_specify=on  socCell_priority=High  socCell=Module19.socCell  socCell_nominal_specify=off  socCell_nominal_value=1  socCell_nominal_unit=1  batteryVoltage_specify=on  batteryVoltage_priority=None  batteryVoltage=Module19.batteryVoltage V  batteryVoltage_nominal_specify=off  batteryVoltage_nominal_value=1  batteryVoltage_nominal_unit=V  batteryCurrent_specify=on  batteryCurrent_priority=None  batteryCurrent=Module19.batteryCurrent A  batteryCurrent_nominal_specify=off  batteryCurrent_nominal_value=1  batteryCurrent_nominal_unit=A  numCycles_specify=on  numCycles_priority=High  numCycles=Module19.numCycles  numCycles_nominal_specify=off  numCycles_nominal_value=1  numCycles_nominal_unit=1  batteryTemperature_specify=on  batteryTemperature_priority=High  batteryTemperature=Module19.batteryTemperature K  batteryTemperature_nominal_specify=off  batteryTemperature_nominal_value=1  batteryTemperature_nominal_unit=K  vParallelAssembly_specify=on  vParallelAssembly_priority=None  vParallelAssembly=Module19.vParallelAssembly V  vParallelAssembly_nominal_specify=off  vParallelAssembly_nominal_value=1  vParallelAssembly_nominal_unit=V  socParallelAssembly_specify=on  socParallelAssembly_priority=None  socParallelAssembly=Module19.socParallelAssembly  socParallelAssembly_nominal_specify=off  socParallelAssembly_nominal_value=1  socParallelAssembly_nominal_unit=1
      settings: InternalSimscapePortConfiguration="{\"Bottom\":[{\"id\":\"n\",\"label\":\"-\",\"type\":\"foundation.electrical.electrical\"}],\"Left\":[{\"id\":\"AmbH\",\"label\":\"AmbH\",\"type\":\"foundation.thermal.thermal\"}],\"Right\":[],\"Top\":[{\"id\":\"p\",\"label\":\"+\",\"type\":\"foundation.electrical.electrical\"}]}"
  Module19_outputs : SimscapeProbe  BoundBlock=20  Variables="{\"batteryCurrent\":{\"Probing\":\"ON\"},\"batteryTemperature\":{\"Probing\":\"ON\"},\"batteryVoltage\":{\"Probing\":\"ON\"},\"numCycles\":{\"Probing\":\"ON\"},\"socCell\":{\"Probing\":\"ON\"},\"socParallelAssembly\":{\"Probing\":\"ON\"},\"vParallelAssembly\":{\"Probing\":\"ON\"}}"
  Module20 : thermalCoupledCellResolution_lib/Modules/ModuleType1  BatteryCapacityCell=Module20.BatteryCapacityCell A*hr  BatteryCapacityCellPercentDeviation=Module20.BatteryCapacityCellPercentDeviation  ExtrapolationMethodCell=simscape.enum.extrapolation.nearest  SOCBreakpointsCell=Module20.SOCBreakpointsCell  SOCBreakpointsCellPercentDeviation=Module20.SOCBreakpointsCellPercentDeviation  TemperatureBreakpointsCell=Module20.TemperatureBreakpointsCell K  TemperatureBreakpointsCellPercentDeviation=Module20.TemperatureBreakpointsCellPercentDeviation  OpenCircuitVoltageThermalCell=Module20.OpenCircuitVoltageThermalCell V  OpenCircuitVoltageThermalCellPercentDeviation=Module20.OpenCircuitVoltageThermalCellPercentDeviation  VoltageRangeCell=Module20.VoltageRangeCell V  VoltageRangeCellPercentDeviation=Module20.VoltageRangeCellPercentDeviation  ResistanceSOCBreakpointsCell=Module20.ResistanceSOCBreakpointsCell  ResistanceSOCBreakpointsCellPercentDeviation=Module20.ResistanceSOCBreakpointsCellPercentDeviation  ResistanceTemperatureBreakpointsCell=Module20.ResistanceTemperatureBreakpointsCell K  ResistanceTemperatureBreakpointsCellPercentDeviation=Module20.ResistanceTemperatureBreakpointsCellPercentDeviation  R0ThermalCell=Module20.R0ThermalCell Ohm  R0ThermalCellPercentDeviation=Module20.R0ThermalCellPercentDeviation  R1ThermalCell=Module20.R1ThermalCell Ohm  R1ThermalCellPercentDeviation=Module20.R1ThermalCellPercentDeviation  Tau1ThermalCell=Module20.Tau1ThermalCell s  Tau1ThermalCellPercentDeviation=Module20.Tau1ThermalCellPercentDeviation  BatteryThermalMassCell=Module20.BatteryThermalMassCell J/K  BatteryThermalMassCellPercentDeviation=Module20.BatteryThermalMassCellPercentDeviation  AmbientResistance=Module20.AmbientResistance K/W  P=2  S=6  socCell_specify=on  socCell_priority=High  socCell=Module20.socCell  socCell_nominal_specify=off  socCell_nominal_value=1  socCell_nominal_unit=1  batteryVoltage_specify=on  batteryVoltage_priority=None  batteryVoltage=Module20.batteryVoltage V  batteryVoltage_nominal_specify=off  batteryVoltage_nominal_value=1  batteryVoltage_nominal_unit=V  batteryCurrent_specify=on  batteryCurrent_priority=None  batteryCurrent=Module20.batteryCurrent A  batteryCurrent_nominal_specify=off  batteryCurrent_nominal_value=1  batteryCurrent_nominal_unit=A  numCycles_specify=on  numCycles_priority=High  numCycles=Module20.numCycles  numCycles_nominal_specify=off  numCycles_nominal_value=1  numCycles_nominal_unit=1  batteryTemperature_specify=on  batteryTemperature_priority=High  batteryTemperature=Module20.batteryTemperature K  batteryTemperature_nominal_specify=off  batteryTemperature_nominal_value=1  batteryTemperature_nominal_unit=K  vParallelAssembly_specify=on  vParallelAssembly_priority=None  vParallelAssembly=Module20.vParallelAssembly V  vParallelAssembly_nominal_specify=off  vParallelAssembly_nominal_value=1  vParallelAssembly_nominal_unit=V  socParallelAssembly_specify=on  socParallelAssembly_priority=None  socParallelAssembly=Module20.socParallelAssembly  socParallelAssembly_nominal_specify=off  socParallelAssembly_nominal_value=1  socParallelAssembly_nominal_unit=1
      settings: InternalSimscapePortConfiguration="{\"Bottom\":[{\"id\":\"n\",\"label\":\"-\",\"type\":\"foundation.electrical.electrical\"}],\"Left\":[{\"id\":\"AmbH\",\"label\":\"AmbH\",\"type\":\"foundation.thermal.thermal\"}],\"Right\":[],\"Top\":[{\"id\":\"p\",\"label\":\"+\",\"type\":\"foundation.electrical.electrical\"}]}"
  Module20_outputs : SimscapeProbe  BoundBlock=21  Variables="{\"batteryCurrent\":{\"Probing\":\"ON\"},\"batteryTemperature\":{\"Probing\":\"ON\"},\"batteryVoltage\":{\"Probing\":\"ON\"},\"numCycles\":{\"Probing\":\"ON\"},\"socCell\":{\"Probing\":\"ON\"},\"socParallelAssembly\":{\"Probing\":\"ON\"},\"vParallelAssembly\":{\"Probing\":\"ON\"}}"
  Module21 : thermalCoupledCellResolution_lib/Modules/ModuleType1  BatteryCapacityCell=Module21.BatteryCapacityCell A*hr  BatteryCapacityCellPercentDeviation=Module21.BatteryCapacityCellPercentDeviation  ExtrapolationMethodCell=simscape.enum.extrapolation.nearest  SOCBreakpointsCell=Module21.SOCBreakpointsCell  SOCBreakpointsCellPercentDeviation=Module21.SOCBreakpointsCellPercentDeviation  TemperatureBreakpointsCell=Module21.TemperatureBreakpointsCell K  TemperatureBreakpointsCellPercentDeviation=Module21.TemperatureBreakpointsCellPercentDeviation  OpenCircuitVoltageThermalCell=Module21.OpenCircuitVoltageThermalCell V  OpenCircuitVoltageThermalCellPercentDeviation=Module21.OpenCircuitVoltageThermalCellPercentDeviation  VoltageRangeCell=Module21.VoltageRangeCell V  VoltageRangeCellPercentDeviation=Module21.VoltageRangeCellPercentDeviation  ResistanceSOCBreakpointsCell=Module21.ResistanceSOCBreakpointsCell  ResistanceSOCBreakpointsCellPercentDeviation=Module21.ResistanceSOCBreakpointsCellPercentDeviation  ResistanceTemperatureBreakpointsCell=Module21.ResistanceTemperatureBreakpointsCell K  ResistanceTemperatureBreakpointsCellPercentDeviation=Module21.ResistanceTemperatureBreakpointsCellPercentDeviation  R0ThermalCell=Module21.R0ThermalCell Ohm  R0ThermalCellPercentDeviation=Module21.R0ThermalCellPercentDeviation  R1ThermalCell=Module21.R1ThermalCell Ohm  R1ThermalCellPercentDeviation=Module21.R1ThermalCellPercentDeviation  Tau1ThermalCell=Module21.Tau1ThermalCell s  Tau1ThermalCellPercentDeviation=Module21.Tau1ThermalCellPercentDeviation  BatteryThermalMassCell=Module21.BatteryThermalMassCell J/K  BatteryThermalMassCellPercentDeviation=Module21.BatteryThermalMassCellPercentDeviation  AmbientResistance=Module21.AmbientResistance K/W  P=2  S=6  socCell_specify=on  socCell_priority=High  socCell=Module21.socCell  socCell_nominal_specify=off  socCell_nominal_value=1  socCell_nominal_unit=1  batteryVoltage_specify=on  batteryVoltage_priority=None  batteryVoltage=Module21.batteryVoltage V  batteryVoltage_nominal_specify=off  batteryVoltage_nominal_value=1  batteryVoltage_nominal_unit=V  batteryCurrent_specify=on  batteryCurrent_priority=None  batteryCurrent=Module21.batteryCurrent A  batteryCurrent_nominal_specify=off  batteryCurrent_nominal_value=1  batteryCurrent_nominal_unit=A  numCycles_specify=on  numCycles_priority=High  numCycles=Module21.numCycles  numCycles_nominal_specify=off  numCycles_nominal_value=1  numCycles_nominal_unit=1  batteryTemperature_specify=on  batteryTemperature_priority=High  batteryTemperature=Module21.batteryTemperature K  batteryTemperature_nominal_specify=off  batteryTemperature_nominal_value=1  batteryTemperature_nominal_unit=K  vParallelAssembly_specify=on  vParallelAssembly_priority=None  vParallelAssembly=Module21.vParallelAssembly V  vParallelAssembly_nominal_specify=off  vParallelAssembly_nominal_value=1  vParallelAssembly_nominal_unit=V  socParallelAssembly_specify=on  socParallelAssembly_priority=None  socParallelAssembly=Module21.socParallelAssembly  socParallelAssembly_nominal_specify=off  socParallelAssembly_nominal_value=1  socParallelAssembly_nominal_unit=1
      settings: InternalSimscapePortConfiguration="{\"Bottom\":[{\"id\":\"n\",\"label\":\"-\",\"type\":\"foundation.electrical.electrical\"}],\"Left\":[{\"id\":\"AmbH\",\"label\":\"AmbH\",\"type\":\"foundation.thermal.thermal\"}],\"Right\":[],\"Top\":[{\"id\":\"p\",\"label\":\"+\",\"type\":\"foundation.electrical.electrical\"}]}"
  Module21_outputs : SimscapeProbe  BoundBlock=22  Variables="{\"batteryCurrent\":{\"Probing\":\"ON\"},\"batteryTemperature\":{\"Probing\":\"ON\"},\"batteryVoltage\":{\"Probing\":\"ON\"},\"numCycles\":{\"Probing\":\"ON\"},\"socCell\":{\"Probing\":\"ON\"},\"socParallelAssembly\":{\"Probing\":\"ON\"},\"vParallelAssembly\":{\"Probing\":\"ON\"}}"
  Module22 : thermalCoupledCellResolution_lib/Modules/ModuleType1  BatteryCapacityCell=Module22.BatteryCapacityCell A*hr  BatteryCapacityCellPercentDeviation=Module22.BatteryCapacityCellPercentDeviation  ExtrapolationMethodCell=simscape.enum.extrapolation.nearest  SOCBreakpointsCell=Module22.SOCBreakpointsCell  SOCBreakpointsCellPercentDeviation=Module22.SOCBreakpointsCellPercentDeviation  TemperatureBreakpointsCell=Module22.TemperatureBreakpointsCell K  TemperatureBreakpointsCellPercentDeviation=Module22.TemperatureBreakpointsCellPercentDeviation  OpenCircuitVoltageThermalCell=Module22.OpenCircuitVoltageThermalCell V  OpenCircuitVoltageThermalCellPercentDeviation=Module22.OpenCircuitVoltageThermalCellPercentDeviation  VoltageRangeCell=Module22.VoltageRangeCell V  VoltageRangeCellPercentDeviation=Module22.VoltageRangeCellPercentDeviation  ResistanceSOCBreakpointsCell=Module22.ResistanceSOCBreakpointsCell  ResistanceSOCBreakpointsCellPercentDeviation=Module22.ResistanceSOCBreakpointsCellPercentDeviation  ResistanceTemperatureBreakpointsCell=Module22.ResistanceTemperatureBreakpointsCell K  ResistanceTemperatureBreakpointsCellPercentDeviation=Module22.ResistanceTemperatureBreakpointsCellPercentDeviation  R0ThermalCell=Module22.R0ThermalCell Ohm  R0ThermalCellPercentDeviation=Module22.R0ThermalCellPercentDeviation  R1ThermalCell=Module22.R1ThermalCell Ohm  R1ThermalCellPercentDeviation=Module22.R1ThermalCellPercentDeviation  Tau1ThermalCell=Module22.Tau1ThermalCell s  Tau1ThermalCellPercentDeviation=Module22.Tau1ThermalCellPercentDeviation  BatteryThermalMassCell=Module22.BatteryThermalMassCell J/K  BatteryThermalMassCellPercentDeviation=Module22.BatteryThermalMassCellPercentDeviation  AmbientResistance=Module22.AmbientResistance K/W  P=2  S=6  socCell_specify=on  socCell_priority=High  socCell=Module22.socCell  socCell_nominal_specify=off  socCell_nominal_value=1  socCell_nominal_unit=1  batteryVoltage_specify=on  batteryVoltage_priority=None  batteryVoltage=Module22.batteryVoltage V  batteryVoltage_nominal_specify=off  batteryVoltage_nominal_value=1  batteryVoltage_nominal_unit=V  batteryCurrent_specify=on  batteryCurrent_priority=None  batteryCurrent=Module22.batteryCurrent A  batteryCurrent_nominal_specify=off  batteryCurrent_nominal_value=1  batteryCurrent_nominal_unit=A  numCycles_specify=on  numCycles_priority=High  numCycles=Module22.numCycles  numCycles_nominal_specify=off  numCycles_nominal_value=1  numCycles_nominal_unit=1  batteryTemperature_specify=on  batteryTemperature_priority=High  batteryTemperature=Module22.batteryTemperature K  batteryTemperature_nominal_specify=off  batteryTemperature_nominal_value=1  batteryTemperature_nominal_unit=K  vParallelAssembly_specify=on  vParallelAssembly_priority=None  vParallelAssembly=Module22.vParallelAssembly V  vParallelAssembly_nominal_specify=off  vParallelAssembly_nominal_value=1  vParallelAssembly_nominal_unit=V  socParallelAssembly_specify=on  socParallelAssembly_priority=None  socParallelAssembly=Module22.socParallelAssembly  socParallelAssembly_nominal_specify=off  socParallelAssembly_nominal_value=1  socParallelAssembly_nominal_unit=1
      settings: InternalSimscapePortConfiguration="{\"Bottom\":[{\"id\":\"n\",\"label\":\"-\",\"type\":\"foundation.electrical.electrical\"}],\"Left\":[{\"id\":\"AmbH\",\"label\":\"AmbH\",\"type\":\"foundation.thermal.thermal\"}],\"Right\":[],\"Top\":[{\"id\":\"p\",\"label\":\"+\",\"type\":\"foundation.electrical.electrical\"}]}"
  Module22_outputs : SimscapeProbe  BoundBlock=23  Variables="{\"batteryCurrent\":{\"Probing\":\"ON\"},\"batteryTemperature\":{\"Probing\":\"ON\"},\"batteryVoltage\":{\"Probing\":\"ON\"},\"numCycles\":{\"Probing\":\"ON\"},\"socCell\":{\"Probing\":\"ON\"},\"socParallelAssembly\":{\"Probing\":\"ON\"},\"vParallelAssembly\":{\"Probing\":\"ON\"}}"
  Module23 : thermalCoupledCellResolution_lib/Modules/ModuleType1  BatteryCapacityCell=Module23.BatteryCapacityCell A*hr  BatteryCapacityCellPercentDeviation=Module23.BatteryCapacityCellPercentDeviation  ExtrapolationMethodCell=simscape.enum.extrapolation.nearest  SOCBreakpointsCell=Module23.SOCBreakpointsCell  SOCBreakpointsCellPercentDeviation=Module23.SOCBreakpointsCellPercentDeviation  TemperatureBreakpointsCell=Module23.TemperatureBreakpointsCell K  TemperatureBreakpointsCellPercentDeviation=Module23.TemperatureBreakpointsCellPercentDeviation  OpenCircuitVoltageThermalCell=Module23.OpenCircuitVoltageThermalCell V  OpenCircuitVoltageThermalCellPercentDeviation=Module23.OpenCircuitVoltageThermalCellPercentDeviation  VoltageRangeCell=Module23.VoltageRangeCell V  VoltageRangeCellPercentDeviation=Module23.VoltageRangeCellPercentDeviation  ResistanceSOCBreakpointsCell=Module23.ResistanceSOCBreakpointsCell  ResistanceSOCBreakpointsCellPercentDeviation=Module23.ResistanceSOCBreakpointsCellPercentDeviation  ResistanceTemperatureBreakpointsCell=Module23.ResistanceTemperatureBreakpointsCell K  ResistanceTemperatureBreakpointsCellPercentDeviation=Module23.ResistanceTemperatureBreakpointsCellPercentDeviation  R0ThermalCell=Module23.R0ThermalCell Ohm  R0ThermalCellPercentDeviation=Module23.R0ThermalCellPercentDeviation  R1ThermalCell=Module23.R1ThermalCell Ohm  R1ThermalCellPercentDeviation=Module23.R1ThermalCellPercentDeviation  Tau1ThermalCell=Module23.Tau1ThermalCell s  Tau1ThermalCellPercentDeviation=Module23.Tau1ThermalCellPercentDeviation  BatteryThermalMassCell=Module23.BatteryThermalMassCell J/K  BatteryThermalMassCellPercentDeviation=Module23.BatteryThermalMassCellPercentDeviation  AmbientResistance=Module23.AmbientResistance K/W  P=2  S=6  socCell_specify=on  socCell_priority=High  socCell=Module23.socCell  socCell_nominal_specify=off  socCell_nominal_value=1  socCell_nominal_unit=1  batteryVoltage_specify=on  batteryVoltage_priority=None  batteryVoltage=Module23.batteryVoltage V  batteryVoltage_nominal_specify=off  batteryVoltage_nominal_value=1  batteryVoltage_nominal_unit=V  batteryCurrent_specify=on  batteryCurrent_priority=None  batteryCurrent=Module23.batteryCurrent A  batteryCurrent_nominal_specify=off  batteryCurrent_nominal_value=1  batteryCurrent_nominal_unit=A  numCycles_specify=on  numCycles_priority=High  numCycles=Module23.numCycles  numCycles_nominal_specify=off  numCycles_nominal_value=1  numCycles_nominal_unit=1  batteryTemperature_specify=on  batteryTemperature_priority=High  batteryTemperature=Module23.batteryTemperature K  batteryTemperature_nominal_specify=off  batteryTemperature_nominal_value=1  batteryTemperature_nominal_unit=K  vParallelAssembly_specify=on  vParallelAssembly_priority=None  vParallelAssembly=Module23.vParallelAssembly V  vParallelAssembly_nominal_specify=off  vParallelAssembly_nominal_value=1  vParallelAssembly_nominal_unit=V  socParallelAssembly_specify=on  socParallelAssembly_priority=None  socParallelAssembly=Module23.socParallelAssembly  socParallelAssembly_nominal_specify=off  socParallelAssembly_nominal_value=1  socParallelAssembly_nominal_unit=1
      settings: InternalSimscapePortConfiguration="{\"Bottom\":[{\"id\":\"n\",\"label\":\"-\",\"type\":\"foundation.electrical.electrical\"}],\"Left\":[{\"id\":\"AmbH\",\"label\":\"AmbH\",\"type\":\"foundation.thermal.thermal\"}],\"Right\":[],\"Top\":[{\"id\":\"p\",\"label\":\"+\",\"type\":\"foundation.electrical.electrical\"}]}"
  Module23_outputs : SimscapeProbe  BoundBlock=24  Variables="{\"batteryCurrent\":{\"Probing\":\"ON\"},\"batteryTemperature\":{\"Probing\":\"ON\"},\"batteryVoltage\":{\"Probing\":\"ON\"},\"numCycles\":{\"Probing\":\"ON\"},\"socCell\":{\"Probing\":\"ON\"},\"socParallelAssembly\":{\"Probing\":\"ON\"},\"vParallelAssembly\":{\"Probing\":\"ON\"}}"
  Module24 : thermalCoupledCellResolution_lib/Modules/ModuleType1  BatteryCapacityCell=Module24.BatteryCapacityCell A*hr  BatteryCapacityCellPercentDeviation=Module24.BatteryCapacityCellPercentDeviation  ExtrapolationMethodCell=simscape.enum.extrapolation.nearest  SOCBreakpointsCell=Module24.SOCBreakpointsCell  SOCBreakpointsCellPercentDeviation=Module24.SOCBreakpointsCellPercentDeviation  TemperatureBreakpointsCell=Module24.TemperatureBreakpointsCell K  TemperatureBreakpointsCellPercentDeviation=Module24.TemperatureBreakpointsCellPercentDeviation  OpenCircuitVoltageThermalCell=Module24.OpenCircuitVoltageThermalCell V  OpenCircuitVoltageThermalCellPercentDeviation=Module24.OpenCircuitVoltageThermalCellPercentDeviation  VoltageRangeCell=Module24.VoltageRangeCell V  VoltageRangeCellPercentDeviation=Module24.VoltageRangeCellPercentDeviation  ResistanceSOCBreakpointsCell=Module24.ResistanceSOCBreakpointsCell  ResistanceSOCBreakpointsCellPercentDeviation=Module24.ResistanceSOCBreakpointsCellPercentDeviation  ResistanceTemperatureBreakpointsCell=Module24.ResistanceTemperatureBreakpointsCell K  ResistanceTemperatureBreakpointsCellPercentDeviation=Module24.ResistanceTemperatureBreakpointsCellPercentDeviation  R0ThermalCell=Module24.R0ThermalCell Ohm  R0ThermalCellPercentDeviation=Module24.R0ThermalCellPercentDeviation  R1ThermalCell=Module24.R1ThermalCell Ohm  R1ThermalCellPercentDeviation=Module24.R1ThermalCellPercentDeviation  Tau1ThermalCell=Module24.Tau1ThermalCell s  Tau1ThermalCellPercentDeviation=Module24.Tau1ThermalCellPercentDeviation  BatteryThermalMassCell=Module24.BatteryThermalMassCell J/K  BatteryThermalMassCellPercentDeviation=Module24.BatteryThermalMassCellPercentDeviation  AmbientResistance=Module24.AmbientResistance K/W  P=2  S=6  socCell_specify=on  socCell_priority=High  socCell=Module24.socCell  socCell_nominal_specify=off  socCell_nominal_value=1  socCell_nominal_unit=1  batteryVoltage_specify=on  batteryVoltage_priority=None  batteryVoltage=Module24.batteryVoltage V  batteryVoltage_nominal_specify=off  batteryVoltage_nominal_value=1  batteryVoltage_nominal_unit=V  batteryCurrent_specify=on  batteryCurrent_priority=None  batteryCurrent=Module24.batteryCurrent A  batteryCurrent_nominal_specify=off  batteryCurrent_nominal_value=1  batteryCurrent_nominal_unit=A  numCycles_specify=on  numCycles_priority=High  numCycles=Module24.numCycles  numCycles_nominal_specify=off  numCycles_nominal_value=1  numCycles_nominal_unit=1  batteryTemperature_specify=on  batteryTemperature_priority=High  batteryTemperature=Module24.batteryTemperature K  batteryTemperature_nominal_specify=off  batteryTemperature_nominal_value=1  batteryTemperature_nominal_unit=K  vParallelAssembly_specify=on  vParallelAssembly_priority=None  vParallelAssembly=Module24.vParallelAssembly V  vParallelAssembly_nominal_specify=off  vParallelAssembly_nominal_value=1  vParallelAssembly_nominal_unit=V  socParallelAssembly_specify=on  socParallelAssembly_priority=None  socParallelAssembly=Module24.socParallelAssembly  socParallelAssembly_nominal_specify=off  socParallelAssembly_nominal_value=1  socParallelAssembly_nominal_unit=1
      settings: InternalSimscapePortConfiguration="{\"Bottom\":[{\"id\":\"n\",\"label\":\"-\",\"type\":\"foundation.electrical.electrical\"}],\"Left\":[{\"id\":\"AmbH\",\"label\":\"AmbH\",\"type\":\"foundation.thermal.thermal\"}],\"Right\":[],\"Top\":[{\"id\":\"p\",\"label\":\"+\",\"type\":\"foundation.electrical.electrical\"}]}"
  Module24_outputs : SimscapeProbe  BoundBlock=25  Variables="{\"batteryCurrent\":{\"Probing\":\"ON\"},\"batteryTemperature\":{\"Probing\":\"ON\"},\"batteryVoltage\":{\"Probing\":\"ON\"},\"numCycles\":{\"Probing\":\"ON\"},\"socCell\":{\"Probing\":\"ON\"},\"socParallelAssembly\":{\"Probing\":\"ON\"},\"vParallelAssembly\":{\"Probing\":\"ON\"}}"
  Module25 : thermalCoupledCellResolution_lib/Modules/ModuleType1  BatteryCapacityCell=Module25.BatteryCapacityCell A*hr  BatteryCapacityCellPercentDeviation=Module25.BatteryCapacityCellPercentDeviation  ExtrapolationMethodCell=simscape.enum.extrapolation.nearest  SOCBreakpointsCell=Module25.SOCBreakpointsCell  SOCBreakpointsCellPercentDeviation=Module25.SOCBreakpointsCellPercentDeviation  TemperatureBreakpointsCell=Module25.TemperatureBreakpointsCell K  TemperatureBreakpointsCellPercentDeviation=Module25.TemperatureBreakpointsCellPercentDeviation  OpenCircuitVoltageThermalCell=Module25.OpenCircuitVoltageThermalCell V  OpenCircuitVoltageThermalCellPercentDeviation=Module25.OpenCircuitVoltageThermalCellPercentDeviation  VoltageRangeCell=Module25.VoltageRangeCell V  VoltageRangeCellPercentDeviation=Module25.VoltageRangeCellPercentDeviation  ResistanceSOCBreakpointsCell=Module25.ResistanceSOCBreakpointsCell  ResistanceSOCBreakpointsCellPercentDeviation=Module25.ResistanceSOCBreakpointsCellPercentDeviation  ResistanceTemperatureBreakpointsCell=Module25.ResistanceTemperatureBreakpointsCell K  ResistanceTemperatureBreakpointsCellPercentDeviation=Module25.ResistanceTemperatureBreakpointsCellPercentDeviation  R0ThermalCell=Module25.R0ThermalCell Ohm  R0ThermalCellPercentDeviation=Module25.R0ThermalCellPercentDeviation  R1ThermalCell=Module25.R1ThermalCell Ohm  R1ThermalCellPercentDeviation=Module25.R1ThermalCellPercentDeviation  Tau1ThermalCell=Module25.Tau1ThermalCell s  Tau1ThermalCellPercentDeviation=Module25.Tau1ThermalCellPercentDeviation  BatteryThermalMassCell=Module25.BatteryThermalMassCell J/K  BatteryThermalMassCellPercentDeviation=Module25.BatteryThermalMassCellPercentDeviation  AmbientResistance=Module25.AmbientResistance K/W  P=2  S=6  socCell_specify=on  socCell_priority=High  socCell=Module25.socCell  socCell_nominal_specify=off  socCell_nominal_value=1  socCell_nominal_unit=1  batteryVoltage_specify=on  batteryVoltage_priority=None  batteryVoltage=Module25.batteryVoltage V  batteryVoltage_nominal_specify=off  batteryVoltage_nominal_value=1  batteryVoltage_nominal_unit=V  batteryCurrent_specify=on  batteryCurrent_priority=None  batteryCurrent=Module25.batteryCurrent A  batteryCurrent_nominal_specify=off  batteryCurrent_nominal_value=1  batteryCurrent_nominal_unit=A  numCycles_specify=on  numCycles_priority=High  numCycles=Module25.numCycles  numCycles_nominal_specify=off  numCycles_nominal_value=1  numCycles_nominal_unit=1  batteryTemperature_specify=on  batteryTemperature_priority=High  batteryTemperature=Module25.batteryTemperature K  batteryTemperature_nominal_specify=off  batteryTemperature_nominal_value=1  batteryTemperature_nominal_unit=K  vParallelAssembly_specify=on  vParallelAssembly_priority=None  vParallelAssembly=Module25.vParallelAssembly V  vParallelAssembly_nominal_specify=off  vParallelAssembly_nominal_value=1  vParallelAssembly_nominal_unit=V  socParallelAssembly_specify=on  socParallelAssembly_priority=None  socParallelAssembly=Module25.socParallelAssembly  socParallelAssembly_nominal_specify=off  socParallelAssembly_nominal_value=1  socParallelAssembly_nominal_unit=1
      settings: InternalSimscapePortConfiguration="{\"Bottom\":[{\"id\":\"n\",\"label\":\"-\",\"type\":\"foundation.electrical.electrical\"}],\"Left\":[{\"id\":\"AmbH\",\"label\":\"AmbH\",\"type\":\"foundation.thermal.thermal\"}],\"Right\":[],\"Top\":[{\"id\":\"p\",\"label\":\"+\",\"type\":\"foundation.electrical.electrical\"}]}"
  Module25_outputs : SimscapeProbe  BoundBlock=26  Variables="{\"batteryCurrent\":{\"Probing\":\"ON\"},\"batteryTemperature\":{\"Probing\":\"ON\"},\"batteryVoltage\":{\"Probing\":\"ON\"},\"numCycles\":{\"Probing\":\"ON\"},\"socCell\":{\"Probing\":\"ON\"},\"socParallelAssembly\":{\"Probing\":\"ON\"},\"vParallelAssembly\":{\"Probing\":\"ON\"}}"
  Module26 : thermalCoupledCellResolution_lib/Modules/ModuleType1  BatteryCapacityCell=Module26.BatteryCapacityCell A*hr  BatteryCapacityCellPercentDeviation=Module26.BatteryCapacityCellPercentDeviation  ExtrapolationMethodCell=simscape.enum.extrapolation.nearest  SOCBreakpointsCell=Module26.SOCBreakpointsCell  SOCBreakpointsCellPercentDeviation=Module26.SOCBreakpointsCellPercentDeviation  TemperatureBreakpointsCell=Module26.TemperatureBreakpointsCell K  TemperatureBreakpointsCellPercentDeviation=Module26.TemperatureBreakpointsCellPercentDeviation  OpenCircuitVoltageThermalCell=Module26.OpenCircuitVoltageThermalCell V  OpenCircuitVoltageThermalCellPercentDeviation=Module26.OpenCircuitVoltageThermalCellPercentDeviation  VoltageRangeCell=Module26.VoltageRangeCell V  VoltageRangeCellPercentDeviation=Module26.VoltageRangeCellPercentDeviation  ResistanceSOCBreakpointsCell=Module26.ResistanceSOCBreakpointsCell  ResistanceSOCBreakpointsCellPercentDeviation=Module26.ResistanceSOCBreakpointsCellPercentDeviation  ResistanceTemperatureBreakpointsCell=Module26.ResistanceTemperatureBreakpointsCell K  ResistanceTemperatureBreakpointsCellPercentDeviation=Module26.ResistanceTemperatureBreakpointsCellPercentDeviation  R0ThermalCell=Module26.R0ThermalCell Ohm  R0ThermalCellPercentDeviation=Module26.R0ThermalCellPercentDeviation  R1ThermalCell=Module26.R1ThermalCell Ohm  R1ThermalCellPercentDeviation=Module26.R1ThermalCellPercentDeviation  Tau1ThermalCell=Module26.Tau1ThermalCell s  Tau1ThermalCellPercentDeviation=Module26.Tau1ThermalCellPercentDeviation  BatteryThermalMassCell=Module26.BatteryThermalMassCell J/K  BatteryThermalMassCellPercentDeviation=Module26.BatteryThermalMassCellPercentDeviation  AmbientResistance=Module26.AmbientResistance K/W  P=2  S=6  socCell_specify=on  socCell_priority=High  socCell=Module26.socCell  socCell_nominal_specify=off  socCell_nominal_value=1  socCell_nominal_unit=1  batteryVoltage_specify=on  batteryVoltage_priority=None  batteryVoltage=Module26.batteryVoltage V  batteryVoltage_nominal_specify=off  batteryVoltage_nominal_value=1  batteryVoltage_nominal_unit=V  batteryCurrent_specify=on  batteryCurrent_priority=None  batteryCurrent=Module26.batteryCurrent A  batteryCurrent_nominal_specify=off  batteryCurrent_nominal_value=1  batteryCurrent_nominal_unit=A  numCycles_specify=on  numCycles_priority=High  numCycles=Module26.numCycles  numCycles_nominal_specify=off  numCycles_nominal_value=1  numCycles_nominal_unit=1  batteryTemperature_specify=on  batteryTemperature_priority=High  batteryTemperature=Module26.batteryTemperature K  batteryTemperature_nominal_specify=off  batteryTemperature_nominal_value=1  batteryTemperature_nominal_unit=K  vParallelAssembly_specify=on  vParallelAssembly_priority=None  vParallelAssembly=Module26.vParallelAssembly V  vParallelAssembly_nominal_specify=off  vParallelAssembly_nominal_value=1  vParallelAssembly_nominal_unit=V  socParallelAssembly_specify=on  socParallelAssembly_priority=None  socParallelAssembly=Module26.socParallelAssembly  socParallelAssembly_nominal_specify=off  socParallelAssembly_nominal_value=1  socParallelAssembly_nominal_unit=1
      settings: InternalSimscapePortConfiguration="{\"Bottom\":[{\"id\":\"n\",\"label\":\"-\",\"type\":\"foundation.electrical.electrical\"}],\"Left\":[{\"id\":\"AmbH\",\"label\":\"AmbH\",\"type\":\"foundation.thermal.thermal\"}],\"Right\":[],\"Top\":[{\"id\":\"p\",\"label\":\"+\",\"type\":\"foundation.electrical.electrical\"}]}"
  Module26_outputs : SimscapeProbe  BoundBlock=27  Variables="{\"batteryCurrent\":{\"Probing\":\"ON\"},\"batteryTemperature\":{\"Probing\":\"ON\"},\"batteryVoltage\":{\"Probing\":\"ON\"},\"numCycles\":{\"Probing\":\"ON\"},\"socCell\":{\"Probing\":\"ON\"},\"socParallelAssembly\":{\"Probing\":\"ON\"},\"vParallelAssembly\":{\"Probing\":\"ON\"}}"
  Module27 : thermalCoupledCellResolution_lib/Modules/ModuleType1  BatteryCapacityCell=Module27.BatteryCapacityCell A*hr  BatteryCapacityCellPercentDeviation=Module27.BatteryCapacityCellPercentDeviation  ExtrapolationMethodCell=simscape.enum.extrapolation.nearest  SOCBreakpointsCell=Module27.SOCBreakpointsCell  SOCBreakpointsCellPercentDeviation=Module27.SOCBreakpointsCellPercentDeviation  TemperatureBreakpointsCell=Module27.TemperatureBreakpointsCell K  TemperatureBreakpointsCellPercentDeviation=Module27.TemperatureBreakpointsCellPercentDeviation  OpenCircuitVoltageThermalCell=Module27.OpenCircuitVoltageThermalCell V  OpenCircuitVoltageThermalCellPercentDeviation=Module27.OpenCircuitVoltageThermalCellPercentDeviation  VoltageRangeCell=Module27.VoltageRangeCell V  VoltageRangeCellPercentDeviation=Module27.VoltageRangeCellPercentDeviation  ResistanceSOCBreakpointsCell=Module27.ResistanceSOCBreakpointsCell  ResistanceSOCBreakpointsCellPercentDeviation=Module27.ResistanceSOCBreakpointsCellPercentDeviation  ResistanceTemperatureBreakpointsCell=Module27.ResistanceTemperatureBreakpointsCell K  ResistanceTemperatureBreakpointsCellPercentDeviation=Module27.ResistanceTemperatureBreakpointsCellPercentDeviation  R0ThermalCell=Module27.R0ThermalCell Ohm  R0ThermalCellPercentDeviation=Module27.R0ThermalCellPercentDeviation  R1ThermalCell=Module27.R1ThermalCell Ohm  R1ThermalCellPercentDeviation=Module27.R1ThermalCellPercentDeviation  Tau1ThermalCell=Module27.Tau1ThermalCell s  Tau1ThermalCellPercentDeviation=Module27.Tau1ThermalCellPercentDeviation  BatteryThermalMassCell=Module27.BatteryThermalMassCell J/K  BatteryThermalMassCellPercentDeviation=Module27.BatteryThermalMassCellPercentDeviation  AmbientResistance=Module27.AmbientResistance K/W  P=2  S=6  socCell_specify=on  socCell_priority=High  socCell=Module27.socCell  socCell_nominal_specify=off  socCell_nominal_value=1  socCell_nominal_unit=1  batteryVoltage_specify=on  batteryVoltage_priority=None  batteryVoltage=Module27.batteryVoltage V  batteryVoltage_nominal_specify=off  batteryVoltage_nominal_value=1  batteryVoltage_nominal_unit=V  batteryCurrent_specify=on  batteryCurrent_priority=None  batteryCurrent=Module27.batteryCurrent A  batteryCurrent_nominal_specify=off  batteryCurrent_nominal_value=1  batteryCurrent_nominal_unit=A  numCycles_specify=on  numCycles_priority=High  numCycles=Module27.numCycles  numCycles_nominal_specify=off  numCycles_nominal_value=1  numCycles_nominal_unit=1  batteryTemperature_specify=on  batteryTemperature_priority=High  batteryTemperature=Module27.batteryTemperature K  batteryTemperature_nominal_specify=off  batteryTemperature_nominal_value=1  batteryTemperature_nominal_unit=K  vParallelAssembly_specify=on  vParallelAssembly_priority=None  vParallelAssembly=Module27.vParallelAssembly V  vParallelAssembly_nominal_specify=off  vParallelAssembly_nominal_value=1  vParallelAssembly_nominal_unit=V  socParallelAssembly_specify=on  socParallelAssembly_priority=None  socParallelAssembly=Module27.socParallelAssembly  socParallelAssembly_nominal_specify=off  socParallelAssembly_nominal_value=1  socParallelAssembly_nominal_unit=1
      settings: InternalSimscapePortConfiguration="{\"Bottom\":[{\"id\":\"n\",\"label\":\"-\",\"type\":\"foundation.electrical.electrical\"}],\"Left\":[{\"id\":\"AmbH\",\"label\":\"AmbH\",\"type\":\"foundation.thermal.thermal\"}],\"Right\":[],\"Top\":[{\"id\":\"p\",\"label\":\"+\",\"type\":\"foundation.electrical.electrical\"}]}"
  Module27_outputs : SimscapeProbe  BoundBlock=28  Variables="{\"batteryCurrent\":{\"Probing\":\"ON\"},\"batteryTemperature\":{\"Probing\":\"ON\"},\"batteryVoltage\":{\"Probing\":\"ON\"},\"numCycles\":{\"Probing\":\"ON\"},\"socCell\":{\"Probing\":\"ON\"},\"socParallelAssembly\":{\"Probing\":\"ON\"},\"vParallelAssembly\":{\"Probing\":\"ON\"}}"
  Module28 : thermalCoupledCellResolution_lib/Modules/ModuleType1  BatteryCapacityCell=Module28.BatteryCapacityCell A*hr  BatteryCapacityCellPercentDeviation=Module28.BatteryCapacityCellPercentDeviation  ExtrapolationMethodCell=simscape.enum.extrapolation.nearest  SOCBreakpointsCell=Module28.SOCBreakpointsCell  SOCBreakpointsCellPercentDeviation=Module28.SOCBreakpointsCellPercentDeviation  TemperatureBreakpointsCell=Module28.TemperatureBreakpointsCell K  TemperatureBreakpointsCellPercentDeviation=Module28.TemperatureBreakpointsCellPercentDeviation  OpenCircuitVoltageThermalCell=Module28.OpenCircuitVoltageThermalCell V  OpenCircuitVoltageThermalCellPercentDeviation=Module28.OpenCircuitVoltageThermalCellPercentDeviation  VoltageRangeCell=Module28.VoltageRangeCell V  VoltageRangeCellPercentDeviation=Module28.VoltageRangeCellPercentDeviation  ResistanceSOCBreakpointsCell=Module28.ResistanceSOCBreakpointsCell  ResistanceSOCBreakpointsCellPercentDeviation=Module28.ResistanceSOCBreakpointsCellPercentDeviation  ResistanceTemperatureBreakpointsCell=Module28.ResistanceTemperatureBreakpointsCell K  ResistanceTemperatureBreakpointsCellPercentDeviation=Module28.ResistanceTemperatureBreakpointsCellPercentDeviation  R0ThermalCell=Module28.R0ThermalCell Ohm  R0ThermalCellPercentDeviation=Module28.R0ThermalCellPercentDeviation  R1ThermalCell=Module28.R1ThermalCell Ohm  R1ThermalCellPercentDeviation=Module28.R1ThermalCellPercentDeviation  Tau1ThermalCell=Module28.Tau1ThermalCell s  Tau1ThermalCellPercentDeviation=Module28.Tau1ThermalCellPercentDeviation  BatteryThermalMassCell=Module28.BatteryThermalMassCell J/K  BatteryThermalMassCellPercentDeviation=Module28.BatteryThermalMassCellPercentDeviation  AmbientResistance=Module28.AmbientResistance K/W  P=2  S=6  socCell_specify=on  socCell_priority=High  socCell=Module28.socCell  socCell_nominal_specify=off  socCell_nominal_value=1  socCell_nominal_unit=1  batteryVoltage_specify=on  batteryVoltage_priority=None  batteryVoltage=Module28.batteryVoltage V  batteryVoltage_nominal_specify=off  batteryVoltage_nominal_value=1  batteryVoltage_nominal_unit=V  batteryCurrent_specify=on  batteryCurrent_priority=None  batteryCurrent=Module28.batteryCurrent A  batteryCurrent_nominal_specify=off  batteryCurrent_nominal_value=1  batteryCurrent_nominal_unit=A  numCycles_specify=on  numCycles_priority=High  numCycles=Module28.numCycles  numCycles_nominal_specify=off  numCycles_nominal_value=1  numCycles_nominal_unit=1  batteryTemperature_specify=on  batteryTemperature_priority=High  batteryTemperature=Module28.batteryTemperature K  batteryTemperature_nominal_specify=off  batteryTemperature_nominal_value=1  batteryTemperature_nominal_unit=K  vParallelAssembly_specify=on  vParallelAssembly_priority=None  vParallelAssembly=Module28.vParallelAssembly V  vParallelAssembly_nominal_specify=off  vParallelAssembly_nominal_value=1  vParallelAssembly_nominal_unit=V  socParallelAssembly_specify=on  socParallelAssembly_priority=None  socParallelAssembly=Module28.socParallelAssembly  socParallelAssembly_nominal_specify=off  socParallelAssembly_nominal_value=1  socParallelAssembly_nominal_unit=1
      settings: InternalSimscapePortConfiguration="{\"Bottom\":[{\"id\":\"n\",\"label\":\"-\",\"type\":\"foundation.electrical.electrical\"}],\"Left\":[{\"id\":\"AmbH\",\"label\":\"AmbH\",\"type\":\"foundation.thermal.thermal\"}],\"Right\":[],\"Top\":[{\"id\":\"p\",\"label\":\"+\",\"type\":\"foundation.electrical.electrical\"}]}"
  Module28_outputs : SimscapeProbe  BoundBlock=29  Variables="{\"batteryCurrent\":{\"Probing\":\"ON\"},\"batteryTemperature\":{\"Probing\":\"ON\"},\"batteryVoltage\":{\"Probing\":\"ON\"},\"numCycles\":{\"Probing\":\"ON\"},\"socCell\":{\"Probing\":\"ON\"},\"socParallelAssembly\":{\"Probing\":\"ON\"},\"vParallelAssembly\":{\"Probing\":\"ON\"}}"
  Module29 : thermalCoupledCellResolution_lib/Modules/ModuleType1  BatteryCapacityCell=Module29.BatteryCapacityCell A*hr  BatteryCapacityCellPercentDeviation=Module29.BatteryCapacityCellPercentDeviation  ExtrapolationMethodCell=simscape.enum.extrapolation.nearest  SOCBreakpointsCell=Module29.SOCBreakpointsCell  SOCBreakpointsCellPercentDeviation=Module29.SOCBreakpointsCellPercentDeviation  TemperatureBreakpointsCell=Module29.TemperatureBreakpointsCell K  TemperatureBreakpointsCellPercentDeviation=Module29.TemperatureBreakpointsCellPercentDeviation  OpenCircuitVoltageThermalCell=Module29.OpenCircuitVoltageThermalCell V  OpenCircuitVoltageThermalCellPercentDeviation=Module29.OpenCircuitVoltageThermalCellPercentDeviation  VoltageRangeCell=Module29.VoltageRangeCell V  VoltageRangeCellPercentDeviation=Module29.VoltageRangeCellPercentDeviation  ResistanceSOCBreakpointsCell=Module29.ResistanceSOCBreakpointsCell  ResistanceSOCBreakpointsCellPercentDeviation=Module29.ResistanceSOCBreakpointsCellPercentDeviation  ResistanceTemperatureBreakpointsCell=Module29.ResistanceTemperatureBreakpointsCell K  ResistanceTemperatureBreakpointsCellPercentDeviation=Module29.ResistanceTemperatureBreakpointsCellPercentDeviation  R0ThermalCell=Module29.R0ThermalCell Ohm  R0ThermalCellPercentDeviation=Module29.R0ThermalCellPercentDeviation  R1ThermalCell=Module29.R1ThermalCell Ohm  R1ThermalCellPercentDeviation=Module29.R1ThermalCellPercentDeviation  Tau1ThermalCell=Module29.Tau1ThermalCell s  Tau1ThermalCellPercentDeviation=Module29.Tau1ThermalCellPercentDeviation  BatteryThermalMassCell=Module29.BatteryThermalMassCell J/K  BatteryThermalMassCellPercentDeviation=Module29.BatteryThermalMassCellPercentDeviation  AmbientResistance=Module29.AmbientResistance K/W  P=2  S=6  socCell_specify=on  socCell_priority=High  socCell=Module29.socCell  socCell_nominal_specify=off  socCell_nominal_value=1  socCell_nominal_unit=1  batteryVoltage_specify=on  batteryVoltage_priority=None  batteryVoltage=Module29.batteryVoltage V  batteryVoltage_nominal_specify=off  batteryVoltage_nominal_value=1  batteryVoltage_nominal_unit=V  batteryCurrent_specify=on  batteryCurrent_priority=None  batteryCurrent=Module29.batteryCurrent A  batteryCurrent_nominal_specify=off  batteryCurrent_nominal_value=1  batteryCurrent_nominal_unit=A  numCycles_specify=on  numCycles_priority=High  numCycles=Module29.numCycles  numCycles_nominal_specify=off  numCycles_nominal_value=1  numCycles_nominal_unit=1  batteryTemperature_specify=on  batteryTemperature_priority=High  batteryTemperature=Module29.batteryTemperature K  batteryTemperature_nominal_specify=off  batteryTemperature_nominal_value=1  batteryTemperature_nominal_unit=K  vParallelAssembly_specify=on  vParallelAssembly_priority=None  vParallelAssembly=Module29.vParallelAssembly V  vParallelAssembly_nominal_specify=off  vParallelAssembly_nominal_value=1  vParallelAssembly_nominal_unit=V  socParallelAssembly_specify=on  socParallelAssembly_priority=None  socParallelAssembly=Module29.socParallelAssembly  socParallelAssembly_nominal_specify=off  socParallelAssembly_nominal_value=1  socParallelAssembly_nominal_unit=1
      settings: InternalSimscapePortConfiguration="{\"Bottom\":[{\"id\":\"n\",\"label\":\"-\",\"type\":\"foundation.electrical.electrical\"}],\"Left\":[{\"id\":\"AmbH\",\"label\":\"AmbH\",\"type\":\"foundation.thermal.thermal\"}],\"Right\":[],\"Top\":[{\"id\":\"p\",\"label\":\"+\",\"type\":\"foundation.electrical.electrical\"}]}"
  Module29_outputs : SimscapeProbe  BoundBlock=30  Variables="{\"batteryCurrent\":{\"Probing\":\"ON\"},\"batteryTemperature\":{\"Probing\":\"ON\"},\"batteryVoltage\":{\"Probing\":\"ON\"},\"numCycles\":{\"Probing\":\"ON\"},\"socCell\":{\"Probing\":\"ON\"},\"socParallelAssembly\":{\"Probing\":\"ON\"},\"vParallelAssembly\":{\"Probing\":\"ON\"}}"
  Module30 : thermalCoupledCellResolution_lib/Modules/ModuleType1  BatteryCapacityCell=Module30.BatteryCapacityCell A*hr  BatteryCapacityCellPercentDeviation=Module30.BatteryCapacityCellPercentDeviation  ExtrapolationMethodCell=simscape.enum.extrapolation.nearest  SOCBreakpointsCell=Module30.SOCBreakpointsCell  SOCBreakpointsCellPercentDeviation=Module30.SOCBreakpointsCellPercentDeviation  TemperatureBreakpointsCell=Module30.TemperatureBreakpointsCell K  TemperatureBreakpointsCellPercentDeviation=Module30.TemperatureBreakpointsCellPercentDeviation  OpenCircuitVoltageThermalCell=Module30.OpenCircuitVoltageThermalCell V  OpenCircuitVoltageThermalCellPercentDeviation=Module30.OpenCircuitVoltageThermalCellPercentDeviation  VoltageRangeCell=Module30.VoltageRangeCell V  VoltageRangeCellPercentDeviation=Module30.VoltageRangeCellPercentDeviation  ResistanceSOCBreakpointsCell=Module30.ResistanceSOCBreakpointsCell  ResistanceSOCBreakpointsCellPercentDeviation=Module30.ResistanceSOCBreakpointsCellPercentDeviation  ResistanceTemperatureBreakpointsCell=Module30.ResistanceTemperatureBreakpointsCell K  ResistanceTemperatureBreakpointsCellPercentDeviation=Module30.ResistanceTemperatureBreakpointsCellPercentDeviation  R0ThermalCell=Module30.R0ThermalCell Ohm  R0ThermalCellPercentDeviation=Module30.R0ThermalCellPercentDeviation  R1ThermalCell=Module30.R1ThermalCell Ohm  R1ThermalCellPercentDeviation=Module30.R1ThermalCellPercentDeviation  Tau1ThermalCell=Module30.Tau1ThermalCell s  Tau1ThermalCellPercentDeviation=Module30.Tau1ThermalCellPercentDeviation  BatteryThermalMassCell=Module30.BatteryThermalMassCell J/K  BatteryThermalMassCellPercentDeviation=Module30.BatteryThermalMassCellPercentDeviation  AmbientResistance=Module30.AmbientResistance K/W  P=2  S=6  socCell_specify=on  socCell_priority=High  socCell=Module30.socCell  socCell_nominal_specify=off  socCell_nominal_value=1  socCell_nominal_unit=1  batteryVoltage_specify=on  batteryVoltage_priority=None  batteryVoltage=Module30.batteryVoltage V  batteryVoltage_nominal_specify=off  batteryVoltage_nominal_value=1  batteryVoltage_nominal_unit=V  batteryCurrent_specify=on  batteryCurrent_priority=None  batteryCurrent=Module30.batteryCurrent A  batteryCurrent_nominal_specify=off  batteryCurrent_nominal_value=1  batteryCurrent_nominal_unit=A  numCycles_specify=on  numCycles_priority=High  numCycles=Module30.numCycles  numCycles_nominal_specify=off  numCycles_nominal_value=1  numCycles_nominal_unit=1  batteryTemperature_specify=on  batteryTemperature_priority=High  batteryTemperature=Module30.batteryTemperature K  batteryTemperature_nominal_specify=off  batteryTemperature_nominal_value=1  batteryTemperature_nominal_unit=K  vParallelAssembly_specify=on  vParallelAssembly_priority=None  vParallelAssembly=Module30.vParallelAssembly V  vParallelAssembly_nominal_specify=off  vParallelAssembly_nominal_value=1  vParallelAssembly_nominal_unit=V  socParallelAssembly_specify=on  socParallelAssembly_priority=None  socParallelAssembly=Module30.socParallelAssembly  socParallelAssembly_nominal_specify=off  socParallelAssembly_nominal_value=1  socParallelAssembly_nominal_unit=1
      settings: InternalSimscapePortConfiguration="{\"Bottom\":[{\"id\":\"n\",\"label\":\"-\",\"type\":\"foundation.electrical.electrical\"}],\"Left\":[{\"id\":\"AmbH\",\"label\":\"AmbH\",\"type\":\"foundation.thermal.thermal\"}],\"Right\":[],\"Top\":[{\"id\":\"p\",\"label\":\"+\",\"type\":\"foundation.electrical.electrical\"}]}"
  Module30_outputs : SimscapeProbe  BoundBlock=31  Variables="{\"batteryCurrent\":{\"Probing\":\"ON\"},\"batteryTemperature\":{\"Probing\":\"ON\"},\"batteryVoltage\":{\"Probing\":\"ON\"},\"numCycles\":{\"Probing\":\"ON\"},\"socCell\":{\"Probing\":\"ON\"},\"socParallelAssembly\":{\"Probing\":\"ON\"},\"vParallelAssembly\":{\"Probing\":\"ON\"}}"
  Module31 : thermalCoupledCellResolution_lib/Modules/ModuleType1  BatteryCapacityCell=Module31.BatteryCapacityCell A*hr  BatteryCapacityCellPercentDeviation=Module31.BatteryCapacityCellPercentDeviation  ExtrapolationMethodCell=simscape.enum.extrapolation.nearest  SOCBreakpointsCell=Module31.SOCBreakpointsCell  SOCBreakpointsCellPercentDeviation=Module31.SOCBreakpointsCellPercentDeviation  TemperatureBreakpointsCell=Module31.TemperatureBreakpointsCell K  TemperatureBreakpointsCellPercentDeviation=Module31.TemperatureBreakpointsCellPercentDeviation  OpenCircuitVoltageThermalCell=Module31.OpenCircuitVoltageThermalCell V  OpenCircuitVoltageThermalCellPercentDeviation=Module31.OpenCircuitVoltageThermalCellPercentDeviation  VoltageRangeCell=Module31.VoltageRangeCell V  VoltageRangeCellPercentDeviation=Module31.VoltageRangeCellPercentDeviation  ResistanceSOCBreakpointsCell=Module31.ResistanceSOCBreakpointsCell  ResistanceSOCBreakpointsCellPercentDeviation=Module31.ResistanceSOCBreakpointsCellPercentDeviation  ResistanceTemperatureBreakpointsCell=Module31.ResistanceTemperatureBreakpointsCell K  ResistanceTemperatureBreakpointsCellPercentDeviation=Module31.ResistanceTemperatureBreakpointsCellPercentDeviation  R0ThermalCell=Module31.R0ThermalCell Ohm  R0ThermalCellPercentDeviation=Module31.R0ThermalCellPercentDeviation  R1ThermalCell=Module31.R1ThermalCell Ohm  R1ThermalCellPercentDeviation=Module31.R1ThermalCellPercentDeviation  Tau1ThermalCell=Module31.Tau1ThermalCell s  Tau1ThermalCellPercentDeviation=Module31.Tau1ThermalCellPercentDeviation  BatteryThermalMassCell=Module31.BatteryThermalMassCell J/K  BatteryThermalMassCellPercentDeviation=Module31.BatteryThermalMassCellPercentDeviation  AmbientResistance=Module31.AmbientResistance K/W  P=2  S=6  socCell_specify=on  socCell_priority=High  socCell=Module31.socCell  socCell_nominal_specify=off  socCell_nominal_value=1  socCell_nominal_unit=1  batteryVoltage_specify=on  batteryVoltage_priority=None  batteryVoltage=Module31.batteryVoltage V  batteryVoltage_nominal_specify=off  batteryVoltage_nominal_value=1  batteryVoltage_nominal_unit=V  batteryCurrent_specify=on  batteryCurrent_priority=None  batteryCurrent=Module31.batteryCurrent A  batteryCurrent_nominal_specify=off  batteryCurrent_nominal_value=1  batteryCurrent_nominal_unit=A  numCycles_specify=on  numCycles_priority=High  numCycles=Module31.numCycles  numCycles_nominal_specify=off  numCycles_nominal_value=1  numCycles_nominal_unit=1  batteryTemperature_specify=on  batteryTemperature_priority=High  batteryTemperature=Module31.batteryTemperature K  batteryTemperature_nominal_specify=off  batteryTemperature_nominal_value=1  batteryTemperature_nominal_unit=K  vParallelAssembly_specify=on  vParallelAssembly_priority=None  vParallelAssembly=Module31.vParallelAssembly V  vParallelAssembly_nominal_specify=off  vParallelAssembly_nominal_value=1  vParallelAssembly_nominal_unit=V  socParallelAssembly_specify=on  socParallelAssembly_priority=None  socParallelAssembly=Module31.socParallelAssembly  socParallelAssembly_nominal_specify=off  socParallelAssembly_nominal_value=1  socParallelAssembly_nominal_unit=1
      settings: InternalSimscapePortConfiguration="{\"Bottom\":[{\"id\":\"n\",\"label\":\"-\",\"type\":\"foundation.electrical.electrical\"}],\"Left\":[{\"id\":\"AmbH\",\"label\":\"AmbH\",\"type\":\"foundation.thermal.thermal\"}],\"Right\":[],\"Top\":[{\"id\":\"p\",\"label\":\"+\",\"type\":\"foundation.electrical.electrical\"}]}"
  Module31_outputs : SimscapeProbe  BoundBlock=32  Variables="{\"batteryCurrent\":{\"Probing\":\"ON\"},\"batteryTemperature\":{\"Probing\":\"ON\"},\"batteryVoltage\":{\"Probing\":\"ON\"},\"numCycles\":{\"Probing\":\"ON\"},\"socCell\":{\"Probing\":\"ON\"},\"socParallelAssembly\":{\"Probing\":\"ON\"},\"vParallelAssembly\":{\"Probing\":\"ON\"}}"
  Module32 : thermalCoupledCellResolution_lib/Modules/ModuleType1  BatteryCapacityCell=Module32.BatteryCapacityCell A*hr  BatteryCapacityCellPercentDeviation=Module32.BatteryCapacityCellPercentDeviation  ExtrapolationMethodCell=simscape.enum.extrapolation.nearest  SOCBreakpointsCell=Module32.SOCBreakpointsCell  SOCBreakpointsCellPercentDeviation=Module32.SOCBreakpointsCellPercentDeviation  TemperatureBreakpointsCell=Module32.TemperatureBreakpointsCell K  TemperatureBreakpointsCellPercentDeviation=Module32.TemperatureBreakpointsCellPercentDeviation  OpenCircuitVoltageThermalCell=Module32.OpenCircuitVoltageThermalCell V  OpenCircuitVoltageThermalCellPercentDeviation=Module32.OpenCircuitVoltageThermalCellPercentDeviation  VoltageRangeCell=Module32.VoltageRangeCell V  VoltageRangeCellPercentDeviation=Module32.VoltageRangeCellPercentDeviation  ResistanceSOCBreakpointsCell=Module32.ResistanceSOCBreakpointsCell  ResistanceSOCBreakpointsCellPercentDeviation=Module32.ResistanceSOCBreakpointsCellPercentDeviation  ResistanceTemperatureBreakpointsCell=Module32.ResistanceTemperatureBreakpointsCell K  ResistanceTemperatureBreakpointsCellPercentDeviation=Module32.ResistanceTemperatureBreakpointsCellPercentDeviation  R0ThermalCell=Module32.R0ThermalCell Ohm  R0ThermalCellPercentDeviation=Module32.R0ThermalCellPercentDeviation  R1ThermalCell=Module32.R1ThermalCell Ohm  R1ThermalCellPercentDeviation=Module32.R1ThermalCellPercentDeviation  Tau1ThermalCell=Module32.Tau1ThermalCell s  Tau1ThermalCellPercentDeviation=Module32.Tau1ThermalCellPercentDeviation  BatteryThermalMassCell=Module32.BatteryThermalMassCell J/K  BatteryThermalMassCellPercentDeviation=Module32.BatteryThermalMassCellPercentDeviation  AmbientResistance=Module32.AmbientResistance K/W  P=2  S=6  socCell_specify=on  socCell_priority=High  socCell=Module32.socCell  socCell_nominal_specify=off  socCell_nominal_value=1  socCell_nominal_unit=1  batteryVoltage_specify=on  batteryVoltage_priority=None  batteryVoltage=Module32.batteryVoltage V  batteryVoltage_nominal_specify=off  batteryVoltage_nominal_value=1  batteryVoltage_nominal_unit=V  batteryCurrent_specify=on  batteryCurrent_priority=None  batteryCurrent=Module32.batteryCurrent A  batteryCurrent_nominal_specify=off  batteryCurrent_nominal_value=1  batteryCurrent_nominal_unit=A  numCycles_specify=on  numCycles_priority=High  numCycles=Module32.numCycles  numCycles_nominal_specify=off  numCycles_nominal_value=1  numCycles_nominal_unit=1  batteryTemperature_specify=on  batteryTemperature_priority=High  batteryTemperature=Module32.batteryTemperature K  batteryTemperature_nominal_specify=off  batteryTemperature_nominal_value=1  batteryTemperature_nominal_unit=K  vParallelAssembly_specify=on  vParallelAssembly_priority=None  vParallelAssembly=Module32.vParallelAssembly V  vParallelAssembly_nominal_specify=off  vParallelAssembly_nominal_value=1  vParallelAssembly_nominal_unit=V  socParallelAssembly_specify=on  socParallelAssembly_priority=None  socParallelAssembly=Module32.socParallelAssembly  socParallelAssembly_nominal_specify=off  socParallelAssembly_nominal_value=1  socParallelAssembly_nominal_unit=1
      settings: InternalSimscapePortConfiguration="{\"Bottom\":[{\"id\":\"n\",\"label\":\"-\",\"type\":\"foundation.electrical.electrical\"}],\"Left\":[{\"id\":\"AmbH\",\"label\":\"AmbH\",\"type\":\"foundation.thermal.thermal\"}],\"Right\":[],\"Top\":[{\"id\":\"p\",\"label\":\"+\",\"type\":\"foundation.electrical.electrical\"}]}"
  Module32_outputs : SimscapeProbe  BoundBlock=33  Variables="{\"batteryCurrent\":{\"Probing\":\"ON\"},\"batteryTemperature\":{\"Probing\":\"ON\"},\"batteryVoltage\":{\"Probing\":\"ON\"},\"numCycles\":{\"Probing\":\"ON\"},\"socCell\":{\"Probing\":\"ON\"},\"socParallelAssembly\":{\"Probing\":\"ON\"},\"vParallelAssembly\":{\"Probing\":\"ON\"}}"
  batteryCurrentMux : Mux  Inputs=32
  batteryTemperatureMux : Mux  Inputs=32
  batteryVoltageMux : Mux  Inputs=32
  numCyclesMux : Mux  Inputs=32
  socCellMux : Mux  Inputs=32
  socParallelAssemblyMux : Mux  Inputs=32
  vParallelAssemblyMux : Mux  Inputs=32
  + : PMIOPort  Side=Left
  - : PMIOPort  Port=2  Side=Right
  AmbH : PMIOPort  Port=3  Side=Right  ConnectionType=Connection: foundation.thermal.thermal
  batteryCurrent : Outport
  batteryTemperature : Outport  Port=2
  batteryVoltage : Outport  Port=3
  numCycles : Outport  Port=4
  socCell : Outport  Port=5
  socParallelAssembly : Outport  Port=6
  vParallelAssembly : Outport  Port=7
  wires:
  Module01_outputs/1 -> [batteryCurrent1]
  batteryCurrentMux/1 -> batteryCurrent/1
  [batteryCurrent1] -> batteryCurrentMux/1
  Module01_outputs/2 -> [batteryTemperature1]
  batteryTemperatureMux/1 -> batteryTemperature/1
  [batteryTemperature1] -> batteryTemperatureMux/1
  Module01_outputs/3 -> [batteryVoltage1]
  batteryVoltageMux/1 -> batteryVoltage/1
  [batteryVoltage1] -> batteryVoltageMux/1
  Module01_outputs/4 -> [numCycles1]
  numCyclesMux/1 -> numCycles/1
  [numCycles1] -> numCyclesMux/1
  Module01_outputs/5 -> [socCell1]
  socCellMux/1 -> socCell/1
  [socCell1] -> socCellMux/1
  Module01_outputs/6 -> [socParallelAssembly1]
  socParallelAssemblyMux/1 -> socParallelAssembly/1
  [socParallelAssembly1] -> socParallelAssemblyMux/1
  Module01_outputs/7 -> [vParallelAssembly1]
  vParallelAssemblyMux/1 -> vParallelAssembly/1
  [vParallelAssembly1] -> vParallelAssemblyMux/1
  Module02_outputs/1 -> [batteryCurrent2]
  [batteryCurrent2] -> batteryCurrentMux/2
  Module02_outputs/2 -> [batteryTemperature2]
  [batteryTemperature2] -> batteryTemperatureMux/2
  Module02_outputs/3 -> [batteryVoltage2]
  [batteryVoltage2] -> batteryVoltageMux/2
  Module02_outputs/4 -> [numCycles2]
  [numCycles2] -> numCyclesMux/2
  Module02_outputs/5 -> [socCell2]
  [socCell2] -> socCellMux/2
  Module02_outputs/6 -> [socParallelAssembly2]
  [socParallelAssembly2] -> socParallelAssemblyMux/2
  Module02_outputs/7 -> [vParallelAssembly2]
  [vParallelAssembly2] -> vParallelAssemblyMux/2
  Module03_outputs/1 -> [batteryCurrent3]
  [batteryCurrent3] -> batteryCurrentMux/3
  Module03_outputs/2 -> [batteryTemperature3]
  [batteryTemperature3] -> batteryTemperatureMux/3
  Module03_outputs/3 -> [batteryVoltage3]
  [batteryVoltage3] -> batteryVoltageMux/3
  Module03_outputs/4 -> [numCycles3]
  [numCycles3] -> numCyclesMux/3
  Module03_outputs/5 -> [socCell3]
  [socCell3] -> socCellMux/3
  Module03_outputs/6 -> [socParallelAssembly3]
  [socParallelAssembly3] -> socParallelAssemblyMux/3
  Module03_outputs/7 -> [vParallelAssembly3]
  [vParallelAssembly3] -> vParallelAssemblyMux/3
  Module04_outputs/1 -> [batteryCurrent4]
  [batteryCurrent4] -> batteryCurrentMux/4
  Module04_outputs/2 -> [batteryTemperature4]
  [batteryTemperature4] -> batteryTemperatureMux/4
  Module04_outputs/3 -> [batteryVoltage4]
  [batteryVoltage4] -> batteryVoltageMux/4
  Module04_outputs/4 -> [numCycles4]
  [numCycles4] -> numCyclesMux/4
  Module04_outputs/5 -> [socCell4]
  [socCell4] -> socCellMux/4
  Module04_outputs/6 -> [socParallelAssembly4]
  [socParallelAssembly4] -> socParallelAssemblyMux/4
  Module04_outputs/7 -> [vParallelAssembly4]
  [vParallelAssembly4] -> vParallelAssemblyMux/4
  Module05_outputs/1 -> [batteryCurrent5]
  [batteryCurrent5] -> batteryCurrentMux/5
  Module05_outputs/2 -> [batteryTemperature5]
  [batteryTemperature5] -> batteryTemperatureMux/5
  Module05_outputs/3 -> [batteryVoltage5]
  [batteryVoltage5] -> batteryVoltageMux/5
  Module05_outputs/4 -> [numCycles5]
  [numCycles5] -> numCyclesMux/5
  Module05_outputs/5 -> [socCell5]
  [socCell5] -> socCellMux/5
  Module05_outputs/6 -> [socParallelAssembly5]
  [socParallelAssembly5] -> socParallelAssemblyMux/5
  Module05_outputs/7 -> [vParallelAssembly5]
  [vParallelAssembly5] -> vParallelAssemblyMux/5
  Module06_outputs/1 -> [batteryCurrent6]
  [batteryCurrent6] -> batteryCurrentMux/6
  Module06_outputs/2 -> [batteryTemperature6]
  [batteryTemperature6] -> batteryTemperatureMux/6
  Module06_outputs/3 -> [batteryVoltage6]
  [batteryVoltage6] -> batteryVoltageMux/6
  Module06_outputs/4 -> [numCycles6]
  [numCycles6] -> numCyclesMux/6
  Module06_outputs/5 -> [socCell6]
  [socCell6] -> socCellMux/6
  Module06_outputs/6 -> [socParallelAssembly6]
  [socParallelAssembly6] -> socParallelAssemblyMux/6
  Module06_outputs/7 -> [vParallelAssembly6]
  [vParallelAssembly6] -> vParallelAssemblyMux/6
  Module07_outputs/1 -> [batteryCurrent7]
  [batteryCurrent7] -> batteryCurrentMux/7
  Module07_outputs/2 -> [batteryTemperature7]
  [batteryTemperature7] -> batteryTemperatureMux/7
  Module07_outputs/3 -> [batteryVoltage7]
  [batteryVoltage7] -> batteryVoltageMux/7
  Module07_outputs/4 -> [numCycles7]
  [numCycles7] -> numCyclesMux/7
  Module07_outputs/5 -> [socCell7]
  [socCell7] -> socCellMux/7
  Module07_outputs/6 -> [socParallelAssembly7]
  [socParallelAssembly7] -> socParallelAssemblyMux/7
  Module07_outputs/7 -> [vParallelAssembly7]
  [vParallelAssembly7] -> vParallelAssemblyMux/7
  Module08_outputs/1 -> [batteryCurrent8]
  [batteryCurrent8] -> batteryCurrentMux/8
  Module08_outputs/2 -> [batteryTemperature8]
  [batteryTemperature8] -> batteryTemperatureMux/8
  Module08_outputs/3 -> [batteryVoltage8]
  [batteryVoltage8] -> batteryVoltageMux/8
  Module08_outputs/4 -> [numCycles8]
  [numCycles8] -> numCyclesMux/8
  Module08_outputs/5 -> [socCell8]
  [socCell8] -> socCellMux/8
  Module08_outputs/6 -> [socParallelAssembly8]
  [socParallelAssembly8] -> socParallelAssemblyMux/8
  Module08_outputs/7 -> [vParallelAssembly8]
  [vParallelAssembly8] -> vParallelAssemblyMux/8
  Module09_outputs/1 -> [batteryCurrent9]
  [batteryCurrent9] -> batteryCurrentMux/9
  Module09_outputs/2 -> [batteryTemperature9]
  [batteryTemperature9] -> batteryTemperatureMux/9
  Module09_outputs/3 -> [batteryVoltage9]
  [batteryVoltage9] -> batteryVoltageMux/9
  Module09_outputs/4 -> [numCycles9]
  [numCycles9] -> numCyclesMux/9
  Module09_outputs/5 -> [socCell9]
  [socCell9] -> socCellMux/9
  Module09_outputs/6 -> [socParallelAssembly9]
  [socParallelAssembly9] -> socParallelAssemblyMux/9
  Module09_outputs/7 -> [vParallelAssembly9]
  [vParallelAssembly9] -> vParallelAssemblyMux/9
  Module10_outputs/1 -> [batteryCurrent10]
  [batteryCurrent10] -> batteryCurrentMux/10
  Module10_outputs/2 -> [batteryTemperature10]
  [batteryTemperature10] -> batteryTemperatureMux/10
  Module10_outputs/3 -> [batteryVoltage10]
  [batteryVoltage10] -> batteryVoltageMux/10
  Module10_outputs/4 -> [numCycles10]
  [numCycles10] -> numCyclesMux/10
  Module10_outputs/5 -> [socCell10]
  [socCell10] -> socCellMux/10
  Module10_outputs/6 -> [socParallelAssembly10]
  [socParallelAssembly10] -> socParallelAssemblyMux/10
  Module10_outputs/7 -> [vParallelAssembly10]
  [vParallelAssembly10] -> vParallelAssemblyMux/10
  Module11_outputs/1 -> [batteryCurrent11]
  [batteryCurrent11] -> batteryCurrentMux/11
  Module11_outputs/2 -> [batteryTemperature11]
  [batteryTemperature11] -> batteryTemperatureMux/11
  Module11_outputs/3 -> [batteryVoltage11]
  [batteryVoltage11] -> batteryVoltageMux/11
  Module11_outputs/4 -> [numCycles11]
  [numCycles11] -> numCyclesMux/11
  Module11_outputs/5 -> [socCell11]
  [socCell11] -> socCellMux/11
  Module11_outputs/6 -> [socParallelAssembly11]
  [socParallelAssembly11] -> socParallelAssemblyMux/11
  Module11_outputs/7 -> [vParallelAssembly11]
  [vParallelAssembly11] -> vParallelAssemblyMux/11
  Module12_outputs/1 -> [batteryCurrent12]
  [batteryCurrent12] -> batteryCurrentMux/12
  Module12_outputs/2 -> [batteryTemperature12]
  [batteryTemperature12] -> batteryTemperatureMux/12
  Module12_outputs/3 -> [batteryVoltage12]
  [batteryVoltage12] -> batteryVoltageMux/12
  Module12_outputs/4 -> [numCycles12]
  [numCycles12] -> numCyclesMux/12
  Module12_outputs/5 -> [socCell12]
  [socCell12] -> socCellMux/12
  Module12_outputs/6 -> [socParallelAssembly12]
  [socParallelAssembly12] -> socParallelAssemblyMux/12
  Module12_outputs/7 -> [vParallelAssembly12]
  [vParallelAssembly12] -> vParallelAssemblyMux/12
  Module13_outputs/1 -> [batteryCurrent13]
  [batteryCurrent13] -> batteryCurrentMux/13
  Module13_outputs/2 -> [batteryTemperature13]
  [batteryTemperature13] -> batteryTemperatureMux/13
  Module13_outputs/3 -> [batteryVoltage13]
  [batteryVoltage13] -> batteryVoltageMux/13
  Module13_outputs/4 -> [numCycles13]
  [numCycles13] -> numCyclesMux/13
  Module13_outputs/5 -> [socCell13]
  [socCell13] -> socCellMux/13
  Module13_outputs/6 -> [socParallelAssembly13]
  [socParallelAssembly13] -> socParallelAssemblyMux/13
  Module13_outputs/7 -> [vParallelAssembly13]
  [vParallelAssembly13] -> vParallelAssemblyMux/13
  Module14_outputs/1 -> [batteryCurrent14]
  [batteryCurrent14] -> batteryCurrentMux/14
  Module14_outputs/2 -> [batteryTemperature14]
  [batteryTemperature14] -> batteryTemperatureMux/14
  Module14_outputs/3 -> [batteryVoltage14]
  [batteryVoltage14] -> batteryVoltageMux/14
  Module14_outputs/4 -> [numCycles14]
  [numCycles14] -> numCyclesMux/14
  Module14_outputs/5 -> [socCell14]
  [socCell14] -> socCellMux/14
  Module14_outputs/6 -> [socParallelAssembly14]
  [socParallelAssembly14] -> socParallelAssemblyMux/14
  Module14_outputs/7 -> [vParallelAssembly14]
  [vParallelAssembly14] -> vParallelAssemblyMux/14
  Module15_outputs/1 -> [batteryCurrent15]
  [batteryCurrent15] -> batteryCurrentMux/15
  Module15_outputs/2 -> [batteryTemperature15]
  [batteryTemperature15] -> batteryTemperatureMux/15
  Module15_outputs/3 -> [batteryVoltage15]
  [batteryVoltage15] -> batteryVoltageMux/15
  Module15_outputs/4 -> [numCycles15]
  [numCycles15] -> numCyclesMux/15
  Module15_outputs/5 -> [socCell15]
  [socCell15] -> socCellMux/15
  Module15_outputs/6 -> [socParallelAssembly15]
  [socParallelAssembly15] -> socParallelAssemblyMux/15
  Module15_outputs/7 -> [vParallelAssembly15]
  [vParallelAssembly15] -> vParallelAssemblyMux/15
  Module16_outputs/1 -> [batteryCurrent16]
  [batteryCurrent16] -> batteryCurrentMux/16
  Module16_outputs/2 -> [batteryTemperature16]
  [batteryTemperature16] -> batteryTemperatureMux/16
  Module16_outputs/3 -> [batteryVoltage16]
  [batteryVoltage16] -> batteryVoltageMux/16
  Module16_outputs/4 -> [numCycles16]
  [numCycles16] -> numCyclesMux/16
  Module16_outputs/5 -> [socCell16]
  [socCell16] -> socCellMux/16
  Module16_outputs/6 -> [socParallelAssembly16]
  [socParallelAssembly16] -> socParallelAssemblyMux/16
  Module16_outputs/7 -> [vParallelAssembly16]
  [vParallelAssembly16] -> vParallelAssemblyMux/16
  Module17_outputs/1 -> [batteryCurrent17]
  [batteryCurrent17] -> batteryCurrentMux/17
  Module17_outputs/2 -> [batteryTemperature17]
  [batteryTemperature17] -> batteryTemperatureMux/17
  Module17_outputs/3 -> [batteryVoltage17]
  [batteryVoltage17] -> batteryVoltageMux/17
  Module17_outputs/4 -> [numCycles17]
  [numCycles17] -> numCyclesMux/17
  Module17_outputs/5 -> [socCell17]
  [socCell17] -> socCellMux/17
  Module17_outputs/6 -> [socParallelAssembly17]
  [socParallelAssembly17] -> socParallelAssemblyMux/17
  Module17_outputs/7 -> [vParallelAssembly17]
  [vParallelAssembly17] -> vParallelAssemblyMux/17
  Module18_outputs/1 -> [batteryCurrent18]
  [batteryCurrent18] -> batteryCurrentMux/18
  Module18_outputs/2 -> [batteryTemperature18]
  [batteryTemperature18] -> batteryTemperatureMux/18
  Module18_outputs/3 -> [batteryVoltage18]
  [batteryVoltage18] -> batteryVoltageMux/18
  Module18_outputs/4 -> [numCycles18]
  [numCycles18] -> numCyclesMux/18
  Module18_outputs/5 -> [socCell18]
  [socCell18] -> socCellMux/18
  Module18_outputs/6 -> [socParallelAssembly18]
  [socParallelAssembly18] -> socParallelAssemblyMux/18
  Module18_outputs/7 -> [vParallelAssembly18]
  [vParallelAssembly18] -> vParallelAssemblyMux/18
  Module19_outputs/1 -> [batteryCurrent19]
  [batteryCurrent19] -> batteryCurrentMux/19
  Module19_outputs/2 -> [batteryTemperature19]
  [batteryTemperature19] -> batteryTemperatureMux/19
  Module19_outputs/3 -> [batteryVoltage19]
  [batteryVoltage19] -> batteryVoltageMux/19
  Module19_outputs/4 -> [numCycles19]
  [numCycles19] -> numCyclesMux/19
  Module19_outputs/5 -> [socCell19]
  [socCell19] -> socCellMux/19
  Module19_outputs/6 -> [socParallelAssembly19]
  [socParallelAssembly19] -> socParallelAssemblyMux/19
  Module19_outputs/7 -> [vParallelAssembly19]
  [vParallelAssembly19] -> vParallelAssemblyMux/19
  Module20_outputs/1 -> [batteryCurrent20]
  [batteryCurrent20] -> batteryCurrentMux/20
  Module20_outputs/2 -> [batteryTemperature20]
  [batteryTemperature20] -> batteryTemperatureMux/20
  Module20_outputs/3 -> [batteryVoltage20]
  [batteryVoltage20] -> batteryVoltageMux/20
  Module20_outputs/4 -> [numCycles20]
  [numCycles20] -> numCyclesMux/20
  Module20_outputs/5 -> [socCell20]
  [socCell20] -> socCellMux/20
  Module20_outputs/6 -> [socParallelAssembly20]
  [socParallelAssembly20] -> socParallelAssemblyMux/20
  Module20_outputs/7 -> [vParallelAssembly20]
  [vParallelAssembly20] -> vParallelAssemblyMux/20
  Module21_outputs/1 -> [batteryCurrent21]
  [batteryCurrent21] -> batteryCurrentMux/21
  Module21_outputs/2 -> [batteryTemperature21]
  [batteryTemperature21] -> batteryTemperatureMux/21
  Module21_outputs/3 -> [batteryVoltage21]
  [batteryVoltage21] -> batteryVoltageMux/21
  Module21_outputs/4 -> [numCycles21]
  [numCycles21] -> numCyclesMux/21
  Module21_outputs/5 -> [socCell21]
  [socCell21] -> socCellMux/21
  Module21_outputs/6 -> [socParallelAssembly21]
  [socParallelAssembly21] -> socParallelAssemblyMux/21
  Module21_outputs/7 -> [vParallelAssembly21]
  [vParallelAssembly21] -> vParallelAssemblyMux/21
  Module22_outputs/1 -> [batteryCurrent22]
  [batteryCurrent22] -> batteryCurrentMux/22
  Module22_outputs/2 -> [batteryTemperature22]
  [batteryTemperature22] -> batteryTemperatureMux/22
  Module22_outputs/3 -> [batteryVoltage22]
